simulink model "kondisi_genset_isolasi"  (R2024b)
settings: Solver=VariableStepAuto  StartTime=0.0  StopTime=10.0  RelTol=1e-3
undefined symbols (not defined in the file): D1, Delta
libraries: spsThreePhaseBreakerLib x36, spsThreePhaseParallelRLCLoadLib x35, spsThreePhaseTransformerTwoWindingsLib x18, spsThreePhasePISectionLineLib x14, spsExcitationSystemLib x13, spsSynchronousMachinepuStandardLib x13, spsGroundLib x4, spsThreePhaseParallelRLCBranchLib x4, spsThreePhaseVIMeasurementLib x4, spspowerguiLib x1
settings Model: Creator=irfan  LastModifiedBy=irfan

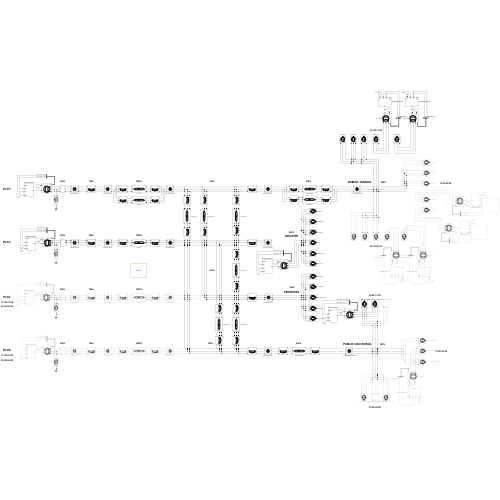
[thumbnail: Simulink's stored preview of the top-level diagram]
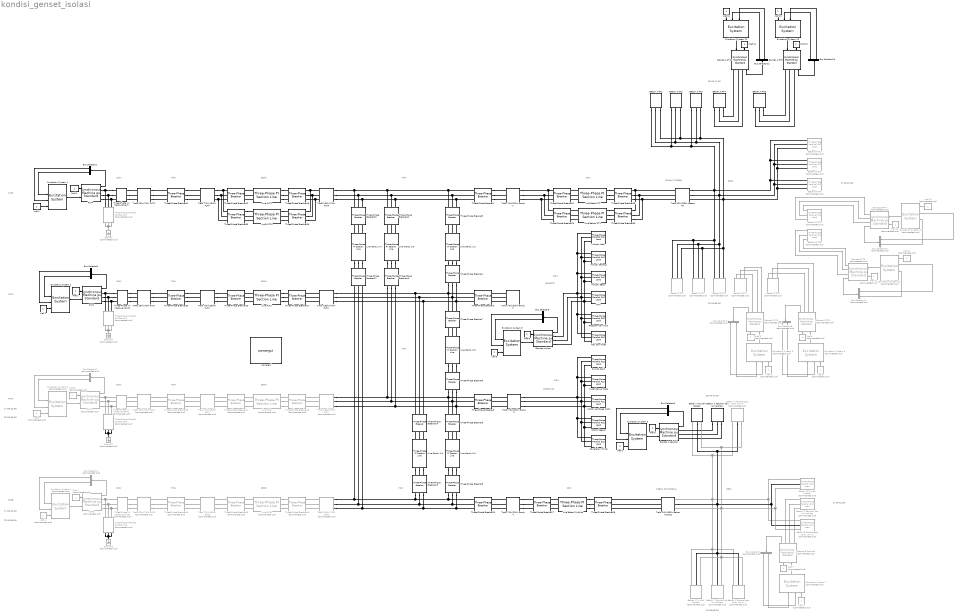
== system kondisi_genset_isolasi ==
  note: 05.00-17.00
  note: PLTP
  note: PLTU
  note: PLTA
  note: PLTB
  note: RUMAH TANGGA
  note: INDUSTRI
  note: PRIORITAS
  note: PUBLIK DAN SOSIAL
  note: 17.00-22.00
  note: 22.00-05.00
  note: 05.00-17.00
  note: 17.00-22.00
  note: 22.00-05.00
  note: 70kV
  note: 150kV
  note: 20kV
  note: 380V
  note: 380V
  note: 17.00-22.00
  note: 17.00-22.00
  note: 20kV
  note: 20kV
  note: 150kV
  note: 150kV
  note: 150kV
  note: 20kV
  note: 70kV
  note: 70kV
  note: 70kV
  note: 70kV
  note: 70kV
  note: 70kV
  note: 20kV
  note: 20kV
  note: 20kV
  note: 20kV
  note: 22.00-05.00
  note: 22.00-05.00
  Beban A Penerangan Jalan Umum : spsThreePhaseParallelRLCLoadLib/Three-Phase Parallel RLC Load  Commented=on  LConnTagsString=A|B|C  Configuration=Y (grounded)  NominalVoltage=380  Vabc=[1e3 1e3 1e3]  Vabcp=[1e3 1e3 1e3]  NominalFrequency=50  UnbalancedPower=off  ActivePower=0e6  InductivePower=0e6  CapacitivePower=0  Pabc=[10e3 9e3 11e3]  QLabc=[100 90 110]  QCabc=[100 90 110]  Pabcp=[10e3 9e3 11e3]  QLabcp=[100 90 110]  QCabcp=[100 90 110]  Measurements=Branch currents  LoadType=constant Z
  Beban A RT1 : spsThreePhaseParallelRLCLoadLib/Three-Phase Parallel RLC Load  LConnTagsString=A|B|C  Configuration=Y (grounded)  NominalVoltage=380  Vabc=[1e3 1e3 1e3]  Vabcp=[1e3 1e3 1e3]  NominalFrequency=50  UnbalancedPower=off  ActivePower=5.1e6  InductivePower=1.68e6  CapacitivePower=0  Pabc=[10e3 9e3 11e3]  QLabc=[100 90 110]  QCabc=[100 90 110]  Pabcp=[10e3 9e3 11e3]  QLabcp=[100 90 110]  QCabcp=[100 90 110]  Measurements=Branch currents  LoadType=constant Z
  Beban A RT2 : spsThreePhaseParallelRLCLoadLib/Three-Phase Parallel RLC Load  LConnTagsString=A|B|C  Configuration=Y (grounded)  NominalVoltage=380  Vabc=[1e3 1e3 1e3]  Vabcp=[1e3 1e3 1e3]  NominalFrequency=50  UnbalancedPower=off  ActivePower=8.06e6  InductivePower=2.65e6  CapacitivePower=0  Pabc=[10e3 9e3 11e3]  QLabc=[100 90 110]  QCabc=[100 90 110]  Pabcp=[10e3 9e3 11e3]  QLabcp=[100 90 110]  QCabcp=[100 90 110]  Measurements=Branch currents  LoadType=constant Z
  Beban A RT3 : spsThreePhaseParallelRLCLoadLib/Three-Phase Parallel RLC Load  LConnTagsString=A|B|C  Configuration=Y (grounded)  NominalVoltage=380  Vabc=[1e3 1e3 1e3]  Vabcp=[1e3 1e3 1e3]  NominalFrequency=50  UnbalancedPower=off  ActivePower=3e6  InductivePower=0.99e6  CapacitivePower=0  Pabc=[10e3 9e3 11e3]  QLabc=[100 90 110]  QCabc=[100 90 110]  Pabcp=[10e3 9e3 11e3]  QLabcp=[100 90 110]  QCabcp=[100 90 110]  Measurements=Branch currents  LoadType=constant Z
  Beban A RT4 : spsThreePhaseParallelRLCLoadLib/Three-Phase Parallel RLC Load  LConnTagsString=A|B|C  Configuration=Y (grounded)  NominalVoltage=380  Vabc=[1e3 1e3 1e3]  Vabcp=[1e3 1e3 1e3]  NominalFrequency=50  UnbalancedPower=off  ActivePower=1.5e6  InductivePower=0.49e6  CapacitivePower=0  Pabc=[10e3 9e3 11e3]  QLabc=[100 90 110]  QCabc=[100 90 110]  Pabcp=[10e3 9e3 11e3]  QLabcp=[100 90 110]  QCabcp=[100 90 110]  Measurements=Branch currents  LoadType=constant Z
  Beban A RT5 : spsThreePhaseParallelRLCLoadLib/Three-Phase Parallel RLC Load  LConnTagsString=A|B|C  Configuration=Y (grounded)  NominalVoltage=380  Vabc=[1e3 1e3 1e3]  Vabcp=[1e3 1e3 1e3]  NominalFrequency=50  UnbalancedPower=off  ActivePower=1.5e6  InductivePower=0.49e6  CapacitivePower=0  Pabc=[10e3 9e3 11e3]  QLabc=[100 90 110]  QCabc=[100 90 110]  Pabcp=[10e3 9e3 11e3]  QLabcp=[100 90 110]  QCabcp=[100 90 110]  Measurements=Branch currents  LoadType=constant Z
  Beban A Rumah Ibadah : spsThreePhaseParallelRLCLoadLib/Three-Phase Parallel RLC Load  LConnTagsString=A|B|C  Configuration=Y (grounded)  NominalVoltage=380  Vabc=[1e3 1e3 1e3]  Vabcp=[1e3 1e3 1e3]  NominalFrequency=50  UnbalancedPower=off  ActivePower=1.122e6  InductivePower=0.6954e6  CapacitivePower=0  Pabc=[10e3 9e3 11e3]  QLabc=[100 90 110]  QCabc=[100 90 110]  Pabcp=[10e3 9e3 11e3]  QLabcp=[100 90 110]  QCabcp=[100 90 110]  Measurements=Branch currents  LoadType=constant Z
  Beban A Sekolah dan Universitas : spsThreePhaseParallelRLCLoadLib/Three-Phase Parallel RLC Load  LConnTagsString=A|B|C  Configuration=Y (grounded)  NominalVoltage=380  Vabc=[1e3 1e3 1e3]  Vabcp=[1e3 1e3 1e3]  NominalFrequency=50  UnbalancedPower=off  ActivePower=0.85e6  InductivePower=0.5268e6  CapacitivePower=0  Pabc=[10e3 9e3 11e3]  QLabc=[100 90 110]  QCabc=[100 90 110]  Pabcp=[10e3 9e3 11e3]  QLabcp=[100 90 110]  QCabcp=[100 90 110]  Measurements=Branch currents  LoadType=constant Z
  Beban B Penerangan Jalan Umum : spsThreePhaseParallelRLCLoadLib/Three-Phase Parallel RLC Load  Commented=on  LConnTagsString=A|B|C  Configuration=Y (grounded)  NominalVoltage=380  Vabc=[1e3 1e3 1e3]  Vabcp=[1e3 1e3 1e3]  NominalFrequency=50  UnbalancedPower=off  ActivePower=1.7e6  InductivePower=1.0536e6  CapacitivePower=0  Pabc=[10e3 9e3 11e3]  QLabc=[100 90 110]  QCabc=[100 90 110]  Pabcp=[10e3 9e3 11e3]  QLabcp=[100 90 110]  QCabcp=[100 90 110]  Measurements=Branch currents  LoadType=constant Z
  Beban B RT1 : spsThreePhaseParallelRLCLoadLib/Three-Phase Parallel RLC Load  Commented=on  LConnTagsString=A|B|C  Configuration=Y (grounded)  NominalVoltage=380  Vabc=[1e3 1e3 1e3]  Vabcp=[1e3 1e3 1e3]  NominalFrequency=50  UnbalancedPower=off  ActivePower=21.93e6  InductivePower=7.21e6  CapacitivePower=0  Pabc=[10e3 9e3 11e3]  QLabc=[100 90 110]  QCabc=[100 90 110]  Pabcp=[10e3 9e3 11e3]  QLabcp=[100 90 110]  QCabcp=[100 90 110]  Measurements=Branch currents  LoadType=constant Z
  Beban B RT2 : spsThreePhaseParallelRLCLoadLib/Three-Phase Parallel RLC Load  Commented=on  LConnTagsString=A|B|C  Configuration=Y (grounded)  NominalVoltage=380  Vabc=[1e3 1e3 1e3]  Vabcp=[1e3 1e3 1e3]  NominalFrequency=50  UnbalancedPower=off  ActivePower=17.58e6  InductivePower=5.78e6  CapacitivePower=0  Pabc=[10e3 9e3 11e3]  QLabc=[100 90 110]  QCabc=[100 90 110]  Pabcp=[10e3 9e3 11e3]  QLabcp=[100 90 110]  QCabcp=[100 90 110]  Measurements=Branch currents  LoadType=constant Z
  Beban B RT3 : spsThreePhaseParallelRLCLoadLib/Three-Phase Parallel RLC Load  Commented=on  LConnTagsString=A|B|C  Configuration=Y (grounded)  NominalVoltage=380  Vabc=[1e3 1e3 1e3]  Vabcp=[1e3 1e3 1e3]  NominalFrequency=50  UnbalancedPower=off  ActivePower=6.53e6  InductivePower=2.14e6  CapacitivePower=0  Pabc=[10e3 9e3 11e3]  QLabc=[100 90 110]  QCabc=[100 90 110]  Pabcp=[10e3 9e3 11e3]  QLabcp=[100 90 110]  QCabcp=[100 90 110]  Measurements=Branch currents  LoadType=constant Z
  Beban B RT4 : spsThreePhaseParallelRLCLoadLib/Three-Phase Parallel RLC Load  Commented=on  LConnTagsString=A|B|C  Configuration=Y (grounded)  NominalVoltage=380  Vabc=[1e3 1e3 1e3]  Vabcp=[1e3 1e3 1e3]  NominalFrequency=50  UnbalancedPower=off  ActivePower=3.26e6  InductivePower=1.07e6  CapacitivePower=0  Pabc=[10e3 9e3 11e3]  QLabc=[100 90 110]  QCabc=[100 90 110]  Pabcp=[10e3 9e3 11e3]  QLabcp=[100 90 110]  QCabcp=[100 90 110]  Measurements=Branch currents  LoadType=constant Z
  Beban B RT5 : spsThreePhaseParallelRLCLoadLib/Three-Phase Parallel RLC Load  Commented=on  LConnTagsString=A|B|C  Configuration=Y (grounded)  NominalVoltage=380  Vabc=[1e3 1e3 1e3]  Vabcp=[1e3 1e3 1e3]  NominalFrequency=50  UnbalancedPower=off  ActivePower=2.91e6  InductivePower=0.96e6  CapacitivePower=0  Pabc=[10e3 9e3 11e3]  QLabc=[100 90 110]  QCabc=[100 90 110]  Pabcp=[10e3 9e3 11e3]  QLabcp=[100 90 110]  QCabcp=[100 90 110]  Measurements=Branch currents  LoadType=constant Z
  Beban B Rumah Ibadah : spsThreePhaseParallelRLCLoadLib/Three-Phase Parallel RLC Load  Commented=on  LConnTagsString=A|B|C  Configuration=Y (grounded)  NominalVoltage=380  Vabc=[1e3 1e3 1e3]  Vabcp=[1e3 1e3 1e3]  NominalFrequency=50  UnbalancedPower=off  ActivePower=1.122e6  InductivePower=0.6954e6  CapacitivePower=0  Pabc=[10e3 9e3 11e3]  QLabc=[100 90 110]  QCabc=[100 90 110]  Pabcp=[10e3 9e3 11e3]  QLabcp=[100 90 110]  QCabcp=[100 90 110]  Measurements=Branch currents  LoadType=constant Z
  Beban B Sekolah dan Universitas : spsThreePhaseParallelRLCLoadLib/Three-Phase Parallel RLC Load  Commented=on  LConnTagsString=A|B|C  Configuration=Y (grounded)  NominalVoltage=380  Vabc=[1e3 1e3 1e3]  Vabcp=[1e3 1e3 1e3]  NominalFrequency=50  UnbalancedPower=off  ActivePower=0.85e6  InductivePower=0.5268e6  CapacitivePower=0  Pabc=[10e3 9e3 11e3]  QLabc=[100 90 110]  QCabc=[100 90 110]  Pabcp=[10e3 9e3 11e3]  QLabcp=[100 90 110]  QCabcp=[100 90 110]  Measurements=Branch currents  LoadType=constant Z
  Beban C Penerangan Jalan Umum : spsThreePhaseParallelRLCLoadLib/Three-Phase Parallel RLC Load  Commented=on  LConnTagsString=A|B|C  Configuration=Y (grounded)  NominalVoltage=380  Vabc=[1e3 1e3 1e3]  Vabcp=[1e3 1e3 1e3]  NominalFrequency=50  UnbalancedPower=off  ActivePower=1.7e6  InductivePower=1.0536e6  CapacitivePower=0  Pabc=[10e3 9e3 11e3]  QLabc=[100 90 110]  QCabc=[100 90 110]  Pabcp=[10e3 9e3 11e3]  QLabcp=[100 90 110]  QCabcp=[100 90 110]  Measurements=Branch currents  LoadType=constant Z
  Beban C RT1 : spsThreePhaseParallelRLCLoadLib/Three-Phase Parallel RLC Load  Commented=on  LConnTagsString=A|B|C  Configuration=Y (grounded)  NominalVoltage=380  Vabc=[1e3 1e3 1e3]  Vabcp=[1e3 1e3 1e3]  NominalFrequency=50  UnbalancedPower=off  ActivePower=15.81e6  InductivePower=5.2e6  CapacitivePower=0  Pabc=[10e3 9e3 11e3]  QLabc=[100 90 110]  QCabc=[100 90 110]  Pabcp=[10e3 9e3 11e3]  QLabcp=[100 90 110]  QCabcp=[100 90 110]  Measurements=Branch currents  LoadType=constant Z
  Beban C RT2 : spsThreePhaseParallelRLCLoadLib/Three-Phase Parallel RLC Load  Commented=on  LConnTagsString=A|B|C  Configuration=Y (grounded)  NominalVoltage=380  Vabc=[1e3 1e3 1e3]  Vabcp=[1e3 1e3 1e3]  NominalFrequency=50  UnbalancedPower=off  ActivePower=13.71e6  InductivePower=4.51e6  CapacitivePower=0  Pabc=[10e3 9e3 11e3]  QLabc=[100 90 110]  QCabc=[100 90 110]  Pabcp=[10e3 9e3 11e3]  QLabcp=[100 90 110]  QCabcp=[100 90 110]  Measurements=Branch currents  LoadType=constant Z
  Beban C RT3 : spsThreePhaseParallelRLCLoadLib/Three-Phase Parallel RLC Load  Commented=on  LConnTagsString=A|B|C  Configuration=Y (grounded)  NominalVoltage=380  Vabc=[1e3 1e3 1e3]  Vabcp=[1e3 1e3 1e3]  NominalFrequency=50  UnbalancedPower=off  ActivePower=5.25e6  InductivePower=1.73e6  CapacitivePower=0  Pabc=[10e3 9e3 11e3]  QLabc=[100 90 110]  QCabc=[100 90 110]  Pabcp=[10e3 9e3 11e3]  QLabcp=[100 90 110]  QCabcp=[100 90 110]  Measurements=Branch currents  LoadType=constant Z
  Beban C RT4 : spsThreePhaseParallelRLCLoadLib/Three-Phase Parallel RLC Load  Commented=on  LConnTagsString=A|B|C  Configuration=Y (grounded)  NominalVoltage=380  Vabc=[1e3 1e3 1e3]  Vabcp=[1e3 1e3 1e3]  NominalFrequency=50  UnbalancedPower=off  ActivePower=2.86e6  InductivePower=0.94e6  CapacitivePower=0  Pabc=[10e3 9e3 11e3]  QLabc=[100 90 110]  QCabc=[100 90 110]  Pabcp=[10e3 9e3 11e3]  QLabcp=[100 90 110]  QCabcp=[100 90 110]  Measurements=Branch currents  LoadType=constant Z
  Beban C RT5 : spsThreePhaseParallelRLCLoadLib/Three-Phase Parallel RLC Load  Commented=on  LConnTagsString=A|B|C  Configuration=Y (grounded)  NominalVoltage=380  Vabc=[1e3 1e3 1e3]  Vabcp=[1e3 1e3 1e3]  NominalFrequency=50  UnbalancedPower=off  ActivePower=3.17e6  InductivePower=1.04e6  CapacitivePower=0  Pabc=[10e3 9e3 11e3]  QLabc=[100 90 110]  QCabc=[100 90 110]  Pabcp=[10e3 9e3 11e3]  QLabcp=[100 90 110]  QCabcp=[100 90 110]  Measurements=Branch currents  LoadType=constant Z
  Beban C Rumah Ibadah : spsThreePhaseParallelRLCLoadLib/Three-Phase Parallel RLC Load  Commented=on  LConnTagsString=A|B|C  Configuration=Y (grounded)  NominalVoltage=380  Vabc=[1e3 1e3 1e3]  Vabcp=[1e3 1e3 1e3]  NominalFrequency=50  UnbalancedPower=off  ActivePower=1.122e6  InductivePower=0.6954e6  CapacitivePower=0  Pabc=[10e3 9e3 11e3]  QLabc=[100 90 110]  QCabc=[100 90 110]  Pabcp=[10e3 9e3 11e3]  QLabcp=[100 90 110]  QCabcp=[100 90 110]  Measurements=Branch currents  LoadType=constant Z
  Beban C Sekolah dan Universitas : spsThreePhaseParallelRLCLoadLib/Three-Phase Parallel RLC Load  Commented=on  LConnTagsString=A|B|C  Configuration=Y (grounded)  NominalVoltage=380  Vabc=[1e3 1e3 1e3]  Vabcp=[1e3 1e3 1e3]  NominalFrequency=50  UnbalancedPower=off  ActivePower=0e6  InductivePower=0e6  CapacitivePower=0  Pabc=[10e3 9e3 11e3]  QLabc=[100 90 110]  QCabc=[100 90 110]  Pabcp=[10e3 9e3 11e3]  QLabcp=[100 90 110]  QCabcp=[100 90 110]  Measurements=Branch currents  LoadType=constant Z
  Bus Selector{1,3,5..6,12..13} (6 alike) : BusSelector  OutputSignals="dq0 components.Stator voltage  vd (pu),dq0 components.Stator voltage  vq (pu)"
  Bus Selector{2,4,7..11} (7 alike) : BusSelector  Commented=on  OutputSignals="dq0 components.Stator voltage  vd (pu),dq0 components.Stator voltage  vq (pu)"
  Excitation System 1 : spsExcitationSystemLib/Excitation System  tr=20e-3  reg=[ 300, 0.001 ]  exc=[ 1, 0 ]  tgr=[ 0, 0 ]  damp=[ 0.001, 0.1 ]  sat=[ 0, 0 ]  lim=[ -11.5, 11.5, 0 ]  v0=[1 2.6645]
      settings: LibrarySourceBlock=sps_lib/Electrical Machines/Synchronous Machine Control/Excitation System
  Excitation System {4,7..11} (6 alike) : spsExcitationSystemLib/Excitation System  Commented=on  tr=20e-3  reg=[ 300, 0.001 ]  exc=[ 1, 0 ]  tgr=[ 0, 0 ]  damp=[ 0.001, 0.1 ]  sat=[ 0, 0 ]  lim=[ -11.5, 11.5, 0 ]  v0=[0.99992 10.989]
      settings: LibrarySourceBlock=sps_lib/Electrical Machines/Synchronous Machine Control/Excitation System
  Excitation System {2,5..6,12..13} (5 alike) : spsExcitationSystemLib/Excitation System  tr=20e-3  reg=[ 300, 0.001 ]  exc=[ 1, 0 ]  tgr=[ 0, 0 ]  damp=[ 0.001, 0.1 ]  sat=[ 0, 0 ]  lim=[ -11.5, 11.5, 0 ]  v0=[0.99992 10.989]
      settings: LibrarySourceBlock=sps_lib/Electrical Machines/Synchronous Machine Control/Excitation System
  Excitation System 3 : spsExcitationSystemLib/Excitation System  Commented=on  tr=20e-3  reg=[ 300, 0.001 ]  exc=[ 1, 0 ]  tgr=[ 0, 0 ]  damp=[ 0.001, 0.1 ]  sat=[ 0, 0 ]  lim=[ -11.5, 11.5, 0 ]  v0=[1 2.6645]
      settings: LibrarySourceBlock=sps_lib/Electrical Machines/Synchronous Machine Control/Excitation System
  Genset A RT4 : spsSynchronousMachinepuStandardLib/Synchronous Machine pu Standard  PresetModel=No  MechanicalLoad=Mechanical power Pm  ShowDetailedParameters=on  RotorType=Salient-pole  Units=per unit standard parameters  MeasurementBus=off  NominalParameters=[1.5789e6 380 50]  Reactances1=[ 1.81, 0.3, 0.23, 1.76, 0.65, 0.25, 0.15 ]  Reactances2=[2.24 0.17 0.12 1.02 0.13 0.1]  dAxisTimeConstants=Short-circuit  qAxisTimeConstants=Short-circuit  TimeConstants1="[ 4.4849  0.0681  0.1  ]"  TimeConstants2=[ 8.0, 0.03, 1.0, 0.07 ]  TimeConstants3="[  4.49  0.0681  0.0513  ]"  TimeConstants4=[ 8.0, 0.03, 0.3371, 0.0295 ]  TimeConstants5=[ 1.01, 0.053, 0.1 ]  TimeConstants6=[ 1.3201, 0.023, 1.0, 0.07 ]  TimeConstants7=[0.012 0.003 0.003]  TimeConstants8=[ 1.3201, 0.0231, 0.3371, 0.0295 ]  StatorResistance=0.037875  Mechanical=[0.1028 0.02056 2]  PolePairs=20  InitialConditions="[ 0  0  0  0  0  0  0  0  1 ]"  SetSaturation=on  Saturation=[0.6404,0.7127,0.8441,0.9214,0.9956,1.082,1.19,1.316,1.457;0.7,0.7698,0.8872,0.9466,0.9969,1.046,1.1,1.151,1.201]  LoadFlowParameters=[1,0,0,0,0]  TsPowergui=0  TsBlock=-1  IterativeModel=Trapezoidal non iterative  IterativeDiscreteModel=Trapezoidal non iterative  BusType=swing  Pref=1.5e6  Qref=0.49e6  Qmin=-inf  Qmax=inf  PLF=0  QLF=0
  Genset A RT5 : spsSynchronousMachinepuStandardLib/Synchronous Machine pu Standard  PresetModel=No  MechanicalLoad=Mechanical power Pm  ShowDetailedParameters=on  RotorType=Salient-pole  Units=per unit standard parameters  MeasurementBus=off  NominalParameters=[1.5789e6 380 50]  Reactances1=[ 1.81, 0.3, 0.23, 1.76, 0.65, 0.25, 0.15 ]  Reactances2=[2.24 0.17 0.12 1.02 0.13 0.1]  dAxisTimeConstants=Short-circuit  qAxisTimeConstants=Short-circuit  TimeConstants1="[ 4.4849  0.0681  0.1  ]"  TimeConstants2=[ 8.0, 0.03, 1.0, 0.07 ]  TimeConstants3="[  4.49  0.0681  0.0513  ]"  TimeConstants4=[ 8.0, 0.03, 0.3371, 0.0295 ]  TimeConstants5=[ 1.01, 0.053, 0.1 ]  TimeConstants6=[ 1.3201, 0.023, 1.0, 0.07 ]  TimeConstants7=[0.012 0.003 0.003]  TimeConstants8=[ 1.3201, 0.0231, 0.3371, 0.0295 ]  StatorResistance=0.037875  Mechanical=[0.1028 0.02056 2]  PolePairs=20  InitialConditions="[ 0  0  0  0  0  0  0  0  1 ]"  SetSaturation=on  Saturation=[0.6404,0.7127,0.8441,0.9214,0.9956,1.082,1.19,1.316,1.457;0.7,0.7698,0.8872,0.9466,0.9969,1.046,1.1,1.151,1.201]  LoadFlowParameters=[1,0,0,0,0]  TsPowergui=0  TsBlock=-1  IterativeModel=Trapezoidal non iterative  IterativeDiscreteModel=Trapezoidal non iterative  BusType=swing  Pref=1.5e6  Qref=0.49e6  Qmin=-inf  Qmax=inf  PLF=0  QLF=0
  Genset A Sekolah : spsSynchronousMachinepuStandardLib/Synchronous Machine pu Standard  PresetModel=No  MechanicalLoad=Mechanical power Pm  ShowDetailedParameters=on  RotorType=Salient-pole  Units=per unit standard parameters  MeasurementBus=off  NominalParameters=[1.0000e6 380 50]  Reactances1=[ 1.81, 0.3, 0.23, 1.76, 0.65, 0.25, 0.15 ]  Reactances2=[2.24 0.17 0.12 1.02 0.13 0.1]  dAxisTimeConstants=Short-circuit  qAxisTimeConstants=Short-circuit  TimeConstants1="[ 4.4849  0.0681  0.1  ]"  TimeConstants2=[ 8.0, 0.03, 1.0, 0.07 ]  TimeConstants3="[  4.49  0.0681  0.0513  ]"  TimeConstants4=[ 8.0, 0.03, 0.3371, 0.0295 ]  TimeConstants5=[ 1.01, 0.053, 0.1 ]  TimeConstants6=[ 1.3201, 0.023, 1.0, 0.07 ]  TimeConstants7=[0.012 0.003 0.003]  TimeConstants8=[ 1.3201, 0.0231, 0.3371, 0.0295 ]  StatorResistance=0.037875  Mechanical=[0.1028 0.02056 2]  PolePairs=20  InitialConditions="[ 0  0  0  0  0  0  0  0  1 ]"  SetSaturation=on  Saturation=[0.6404,0.7127,0.8441,0.9214,0.9956,1.082,1.19,1.316,1.457;0.7,0.7698,0.8872,0.9466,0.9969,1.046,1.1,1.151,1.201]  LoadFlowParameters=[1,0,0,0,0]  TsPowergui=0  TsBlock=-1  IterativeModel=Trapezoidal non iterative  IterativeDiscreteModel=Trapezoidal non iterative  BusType=swing  Pref=0.85e6  Qref=0.5268e6  Qmin=-inf  Qmax=inf  PLF=0  QLF=0
  Genset B RT4 : spsSynchronousMachinepuStandardLib/Synchronous Machine pu Standard  Commented=on  PresetModel=No  MechanicalLoad=Mechanical power Pm  ShowDetailedParameters=on  RotorType=Salient-pole  Units=per unit standard parameters  MeasurementBus=off  NominalParameters=[3.4342e6 380 50]  Reactances1=[ 1.81, 0.3, 0.23, 1.76, 0.65, 0.25, 0.15 ]  Reactances2=[2.24 0.17 0.12 1.02 0.13 0.1]  dAxisTimeConstants=Short-circuit  qAxisTimeConstants=Short-circuit  TimeConstants1="[ 4.4849  0.0681  0.1  ]"  TimeConstants2=[ 8.0, 0.03, 1.0, 0.07 ]  TimeConstants3="[  4.49  0.0681  0.0513  ]"  TimeConstants4=[ 8.0, 0.03, 0.3371, 0.0295 ]  TimeConstants5=[ 1.01, 0.053, 0.1 ]  TimeConstants6=[ 1.3201, 0.023, 1.0, 0.07 ]  TimeConstants7=[0.012 0.003 0.003]  TimeConstants8=[ 1.3201, 0.0231, 0.3371, 0.0295 ]  StatorResistance=0.037875  Mechanical=[0.1028 0.02056 2]  PolePairs=20  InitialConditions="[ 0  0  0  0  0  0  0  0  1 ]"  SetSaturation=on  Saturation=[0.6404,0.7127,0.8441,0.9214,0.9956,1.082,1.19,1.316,1.457;0.7,0.7698,0.8872,0.9466,0.9969,1.046,1.1,1.151,1.201]  LoadFlowParameters=[1,0,0,0,0]  TsPowergui=0  TsBlock=-1  IterativeModel=Trapezoidal non iterative  IterativeDiscreteModel=Trapezoidal non iterative  BusType=swing  Pref=3.26e6  Qref=1.07e6  Qmin=-inf  Qmax=inf  PLF=0  QLF=0
  Genset B RT5 : spsSynchronousMachinepuStandardLib/Synchronous Machine pu Standard  Commented=on  PresetModel=No  MechanicalLoad=Mechanical power Pm  ShowDetailedParameters=on  RotorType=Salient-pole  Units=per unit standard parameters  MeasurementBus=off  NominalParameters=[3.0632e6 380 50]  Reactances1=[ 1.81, 0.3, 0.23, 1.76, 0.65, 0.25, 0.15 ]  Reactances2=[2.24 0.17 0.12 1.02 0.13 0.1]  dAxisTimeConstants=Short-circuit  qAxisTimeConstants=Short-circuit  TimeConstants1="[ 4.4849  0.0681  0.1  ]"  TimeConstants2=[ 8.0, 0.03, 1.0, 0.07 ]  TimeConstants3="[  4.49  0.0681  0.0513  ]"  TimeConstants4=[ 8.0, 0.03, 0.3371, 0.0295 ]  TimeConstants5=[ 1.01, 0.053, 0.1 ]  TimeConstants6=[ 1.3201, 0.023, 1.0, 0.07 ]  TimeConstants7=[0.012 0.003 0.003]  TimeConstants8=[ 1.3201, 0.0231, 0.3371, 0.0295 ]  StatorResistance=0.037875  Mechanical=[0.1028 0.02056 2]  PolePairs=20  InitialConditions="[ 0  0  0  0  0  0  0  0  1 ]"  SetSaturation=on  Saturation=[0.6404,0.7127,0.8441,0.9214,0.9956,1.082,1.19,1.316,1.457;0.7,0.7698,0.8872,0.9466,0.9969,1.046,1.1,1.151,1.201]  LoadFlowParameters=[1,0,0,0,0]  TsPowergui=0  TsBlock=-1  IterativeModel=Trapezoidal non iterative  IterativeDiscreteModel=Trapezoidal non iterative  BusType=swing  Pref=2.91e6  Qref=0.96e6  Qmin=-inf  Qmax=inf  PLF=0  QLF=0
  Genset B Sekolah : spsSynchronousMachinepuStandardLib/Synchronous Machine pu Standard  Commented=on  PresetModel=No  MechanicalLoad=Mechanical power Pm  ShowDetailedParameters=on  RotorType=Salient-pole  Units=per unit standard parameters  MeasurementBus=off  NominalParameters=[1e6 380 50]  Reactances1=[ 1.81, 0.3, 0.23, 1.76, 0.65, 0.25, 0.15 ]  Reactances2=[2.24 0.17 0.12 1.02 0.13 0.1]  dAxisTimeConstants=Short-circuit  qAxisTimeConstants=Short-circuit  TimeConstants1="[ 4.4849  0.0681  0.1  ]"  TimeConstants2=[ 8.0, 0.03, 1.0, 0.07 ]  TimeConstants3="[  4.49  0.0681  0.0513  ]"  TimeConstants4=[ 8.0, 0.03, 0.3371, 0.0295 ]  TimeConstants5=[ 1.01, 0.053, 0.1 ]  TimeConstants6=[ 1.3201, 0.023, 1.0, 0.07 ]  TimeConstants7=[0.012 0.003 0.003]  TimeConstants8=[ 1.3201, 0.0231, 0.3371, 0.0295 ]  StatorResistance=0.037875  Mechanical=[0.1028 0.02056 2]  PolePairs=20  InitialConditions="[ 0  0  0  0  0  0  0  0  1 ]"  SetSaturation=on  Saturation=[0.6404,0.7127,0.8441,0.9214,0.9956,1.082,1.19,1.316,1.457;0.7,0.7698,0.8872,0.9466,0.9969,1.046,1.1,1.151,1.201]  LoadFlowParameters=[1,0,0,0,0]  TsPowergui=0  TsBlock=-1  IterativeModel=Trapezoidal non iterative  IterativeDiscreteModel=Trapezoidal non iterative  BusType=swing  Pref=0.85e6  Qref=0.5268e6  Qmin=-inf  Qmax=inf  PLF=0  QLF=0
  Genset C RT4 : spsSynchronousMachinepuStandardLib/Synchronous Machine pu Standard  Commented=on  PresetModel=No  MechanicalLoad=Mechanical power Pm  ShowDetailedParameters=on  RotorType=Salient-pole  Units=per unit standard parameters  MeasurementBus=off  NominalParameters=[3.0132e6 380 50]  Reactances1=[ 1.81, 0.3, 0.23, 1.76, 0.65, 0.25, 0.15 ]  Reactances2=[2.24 0.17 0.12 1.02 0.13 0.1]  dAxisTimeConstants=Short-circuit  qAxisTimeConstants=Short-circuit  TimeConstants1="[ 4.4849  0.0681  0.1  ]"  TimeConstants2=[ 8.0, 0.03, 1.0, 0.07 ]  TimeConstants3="[  4.49  0.0681  0.0513  ]"  TimeConstants4=[ 8.0, 0.03, 0.3371, 0.0295 ]  TimeConstants5=[ 1.01, 0.053, 0.1 ]  TimeConstants6=[ 1.3201, 0.023, 1.0, 0.07 ]  TimeConstants7=[0.012 0.003 0.003]  TimeConstants8=[ 1.3201, 0.0231, 0.3371, 0.0295 ]  StatorResistance=0.037875  Mechanical=[0.1028 0.02056 2]  PolePairs=20  InitialConditions="[ 0  0  0  0  0  0  0  0  1 ]"  SetSaturation=on  Saturation=[0.6404,0.7127,0.8441,0.9214,0.9956,1.082,1.19,1.316,1.457;0.7,0.7698,0.8872,0.9466,0.9969,1.046,1.1,1.151,1.201]  LoadFlowParameters=[1,0,0,0,0]  TsPowergui=0  TsBlock=-1  IterativeModel=Trapezoidal non iterative  IterativeDiscreteModel=Trapezoidal non iterative  BusType=swing  Pref=2.86e6  Qref=0.94e6  Qmin=-inf  Qmax=inf  PLF=0  QLF=0
  Genset C RT5 : spsSynchronousMachinepuStandardLib/Synchronous Machine pu Standard  Commented=on  PresetModel=No  MechanicalLoad=Mechanical power Pm  ShowDetailedParameters=on  RotorType=Salient-pole  Units=per unit standard parameters  MeasurementBus=off  NominalParameters=[3.3316e6 380 50]  Reactances1=[ 1.81, 0.3, 0.23, 1.76, 0.65, 0.25, 0.15 ]  Reactances2=[2.24 0.17 0.12 1.02 0.13 0.1]  dAxisTimeConstants=Short-circuit  qAxisTimeConstants=Short-circuit  TimeConstants1="[ 4.4849  0.0681  0.1  ]"  TimeConstants2=[ 8.0, 0.03, 1.0, 0.07 ]  TimeConstants3="[  4.49  0.0681  0.0513  ]"  TimeConstants4=[ 8.0, 0.03, 0.3371, 0.0295 ]  TimeConstants5=[ 1.01, 0.053, 0.1 ]  TimeConstants6=[ 1.3201, 0.023, 1.0, 0.07 ]  TimeConstants7=[0.012 0.003 0.003]  TimeConstants8=[ 1.3201, 0.0231, 0.3371, 0.0295 ]  StatorResistance=0.037875  Mechanical=[0.1028 0.02056 2]  PolePairs=20  InitialConditions="[ 0  0  0  0  0  0  0  0  1 ]"  SetSaturation=on  Saturation=[0.6404,0.7127,0.8441,0.9214,0.9956,1.082,1.19,1.316,1.457;0.7,0.7698,0.8872,0.9466,0.9969,1.046,1.1,1.151,1.201]  LoadFlowParameters=[1,0,0,0,0]  TsPowergui=0  TsBlock=-1  IterativeModel=Trapezoidal non iterative  IterativeDiscreteModel=Trapezoidal non iterative  BusType=swing  Pref=3.17e6  Qref=1.04e6  Qmin=-inf  Qmax=inf  PLF=0  QLF=0
  Genset Industri : spsSynchronousMachinepuStandardLib/Synchronous Machine pu Standard  PresetModel=No  MechanicalLoad=Mechanical power Pm  ShowDetailedParameters=on  RotorType=Salient-pole  Units=per unit standard parameters  MeasurementBus=off  NominalParameters=[79.1000e6 20e3 50]  Reactances1=[ 1.81, 0.3, 0.23, 1.76, 0.65, 0.25, 0.15 ]  Reactances2=[2.24 0.17 0.12 1.02 0.13 0.1]  dAxisTimeConstants=Short-circuit  qAxisTimeConstants=Short-circuit  TimeConstants1="[ 4.4849  0.0681  0.1  ]"  TimeConstants2=[ 8.0, 0.03, 1.0, 0.07 ]  TimeConstants3="[  4.49  0.0681  0.0513  ]"  TimeConstants4=[ 8.0, 0.03, 0.3371, 0.0295 ]  TimeConstants5=[ 1.01, 0.053, 0.1 ]  TimeConstants6=[ 1.3201, 0.023, 1.0, 0.07 ]  TimeConstants7=[0.012 0.003 0.003]  TimeConstants8=[ 1.3201, 0.0231, 0.3371, 0.0295 ]  StatorResistance=0.037875  Mechanical=[0.1028 0.02056 2]  PolePairs=20  InitialConditions="[ 0  0  0  0  0  0  0  0  1 ]"  SetSaturation=on  Saturation=[0.6404,0.7127,0.8441,0.9214,0.9956,1.082,1.19,1.316,1.457;0.7,0.7698,0.8872,0.9466,0.9969,1.046,1.1,1.151,1.201]  LoadFlowParameters=[1,0,0,0,0]  TsPowergui=0  TsBlock=-1  IterativeModel=Trapezoidal non iterative  IterativeDiscreteModel=Trapezoidal non iterative  BusType=swing  Pref=71.248e6  Qref=34.0616e6  Qmin=-inf  Qmax=inf  PLF=0  QLF=0
  Ground{,1..3} (4 alike) : spsGroundLib/Ground  Commented=on  LConnTagsString=a
  Industri Besar : spsThreePhaseParallelRLCLoadLib/Three-Phase Parallel RLC Load  LConnTagsString=A|B|C  Configuration=Y (grounded)  NominalVoltage=20e3  Vabc=[1e3 1e3 1e3]  Vabcp=[1e3 1e3 1e3]  NominalFrequency=50  UnbalancedPower=off  ActivePower=9.5e6  InductivePower=3.1225e6  CapacitivePower=0  Pabc=[10e3 9e3 11e3]  QLabc=[100 90 110]  QCabc=[100 90 110]  Pabcp=[10e3 9e3 11e3]  QLabcp=[100 90 110]  QCabcp=[100 90 110]  Measurements=Branch currents  LoadType=constant Z
  Industri Kecil : spsThreePhaseParallelRLCLoadLib/Three-Phase Parallel RLC Load  LConnTagsString=A|B|C  Configuration=Y (grounded)  NominalVoltage=20e3  Vabc=[1e3 1e3 1e3]  Vabcp=[1e3 1e3 1e3]  NominalFrequency=50  UnbalancedPower=off  ActivePower=5.808e6  InductivePower=3.1348e6  CapacitivePower=0  Pabc=[10e3 9e3 11e3]  QLabc=[100 90 110]  QCabc=[100 90 110]  Pabcp=[10e3 9e3 11e3]  QLabcp=[100 90 110]  QCabcp=[100 90 110]  Measurements=Branch currents  LoadType=constant Z
  Industri Sedang : spsThreePhaseParallelRLCLoadLib/Three-Phase Parallel RLC Load  LConnTagsString=A|B|C  Configuration=Y (grounded)  NominalVoltage=20e3  Vabc=[1e3 1e3 1e3]  Vabcp=[1e3 1e3 1e3]  NominalFrequency=50  UnbalancedPower=off  ActivePower=45e6  InductivePower=21.7945e6  CapacitivePower=0  Pabc=[10e3 9e3 11e3]  QLabc=[100 90 110]  QCabc=[100 90 110]  Pabcp=[10e3 9e3 11e3]  QLabcp=[100 90 110]  QCabcp=[100 90 110]  Measurements=Branch currents  LoadType=constant Z
  Istana Negara : spsThreePhaseParallelRLCLoadLib/Three-Phase Parallel RLC Load  LConnTagsString=A|B|C  Configuration=Y (grounded)  NominalVoltage=20e3  Vabc=[1e3 1e3 1e3]  Vabcp=[1e3 1e3 1e3]  NominalFrequency=50  UnbalancedPower=off  ActivePower=0.9e6  InductivePower=0.4359e6  CapacitivePower=0  Pabc=[10e3 9e3 11e3]  QLabc=[100 90 110]  QCabc=[100 90 110]  Pabcp=[10e3 9e3 11e3]  QLabcp=[100 90 110]  QCabcp=[100 90 110]  Measurements=Branch currents  LoadType=constant Z
  Kantor Lembaga Data : spsThreePhaseParallelRLCLoadLib/Three-Phase Parallel RLC Load  LConnTagsString=A|B|C  Configuration=Y (grounded)  NominalVoltage=20e3  Vabc=[1e3 1e3 1e3]  Vabcp=[1e3 1e3 1e3]  NominalFrequency=50  UnbalancedPower=off  ActivePower=0.9e6  InductivePower=0.4359e6  CapacitivePower=0  Pabc=[10e3 9e3 11e3]  QLabc=[100 90 110]  QCabc=[100 90 110]  Pabcp=[10e3 9e3 11e3]  QLabcp=[100 90 110]  QCabcp=[100 90 110]  Measurements=Branch currents  LoadType=constant Z
  Line Beban PubSos : spsThreePhasePISectionLineLib/Three-Phase PI Section Line  LConnTagsString=a|b|c  RConnTagsString=A|B|C  Length=3  Frequency=50  Resistances=[ 0.2530 0.3864]  Inductances="[ 0.5530e-3  4.1264e-3]"  Capacitances=[0.2060e-6 7.751e-9]
  Line Beban RT : spsThreePhasePISectionLineLib/Three-Phase PI Section Line  LConnTagsString=a|b|c  RConnTagsString=A|B|C  Length=3  Frequency=50  Resistances=[ 0.2530 0.3864]  Inductances="[ 0.5530e-3  4.1264e-3]"  Capacitances=[0.2060e-6 7.751e-9]
  Line Beban RT1 : spsThreePhasePISectionLineLib/Three-Phase PI Section Line  LConnTagsString=a|b|c  RConnTagsString=A|B|C  Length=3  Frequency=50  Resistances=[ 0.2530 0.3864]  Inductances="[ 0.5530e-3  4.1264e-3]"  Capacitances=[0.2060e-6 7.751e-9]
  Line Gardu 1-2 : spsThreePhasePISectionLineLib/Three-Phase PI Section Line  LConnTagsString=a|b|c  RConnTagsString=A|B|C  Length=20  Frequency=50  Resistances=[ 0.0605 0.3864]  Inductances="[ 0.6210e-3  4.1264e-3]"  Capacitances=[12.74e-9 7.751e-9]
  Line Gardu 1-3 : spsThreePhasePISectionLineLib/Three-Phase PI Section Line  LConnTagsString=a|b|c  RConnTagsString=A|B|C  Length=5  Frequency=50  Resistances=[ 0.0605 0.3864]  Inductances="[ 0.6210e-3  4.1264e-3]"  Capacitances=[12.74e-9 7.751e-9]
  Line Gardu 1-4 : spsThreePhasePISectionLineLib/Three-Phase PI Section Line  LConnTagsString=a|b|c  RConnTagsString=A|B|C  Length=20  Frequency=50  Resistances=[ 0.0605 0.3864]  Inductances="[ 0.6210e-3  4.1264e-3]"  Capacitances=[12.74e-9 7.751e-9]
  Line Gardu 2-3 : spsThreePhasePISectionLineLib/Three-Phase PI Section Line  LConnTagsString=a|b|c  RConnTagsString=A|B|C  Length=5  Frequency=50  Resistances=[ 0.0605 0.3864]  Inductances="[ 0.6210e-3  4.1264e-3]"  Capacitances=[12.74e-9 7.751e-9]
  Line Gardu 2-4 : spsThreePhasePISectionLineLib/Three-Phase PI Section Line  LConnTagsString=a|b|c  RConnTagsString=A|B|C  Length=20  Frequency=50  Resistances=[ 0.0605 0.3864]  Inductances="[ 0.0012  0.0035]"  Capacitances=[12.74e-9 7.751e-9]
  Line Gardu 3-4 : spsThreePhasePISectionLineLib/Three-Phase PI Section Line  LConnTagsString=a|b|c  RConnTagsString=A|B|C  Length=5  Frequency=50  Resistances=[ 0.0605 0.3864]  Inductances="[ 0.6210e-3  4.1264e-3]"  Capacitances=[12.74e-9 7.751e-9]
  Line PLTA : spsThreePhasePISectionLineLib/Three-Phase PI Section Line  Commented=on  LConnTagsString=a|b|c  RConnTagsString=A|B|C  Length=50  Frequency=50  Resistances=[ 0.0605 0.3864]  Inductances="[ 0.6210e-3  4.1264e-3]"  Capacitances=[12.74e-9 7.751e-9]
  Line PLTB : spsThreePhasePISectionLineLib/Three-Phase PI Section Line  Commented=on  LConnTagsString=a|b|c  RConnTagsString=A|B|C  Length=20  Frequency=50  Resistances=[ 0.0605 0.3864]  Inductances="[ 0.6210e-3  4.1264e-3]"  Capacitances=[0.149e-6 5e-9]
  Line PLTP : spsThreePhasePISectionLineLib/Three-Phase PI Section Line  LConnTagsString=a|b|c  RConnTagsString=A|B|C  Length=100  Frequency=50  Resistances=[ 0.0605 0.3864]  Inductances="[ 0.6210e-3  4.1264e-3]"  Capacitances=[12.74e-9 7.751e-9]
  Line PLTP1 : spsThreePhasePISectionLineLib/Three-Phase PI Section Line  LConnTagsString=a|b|c  RConnTagsString=A|B|C  Length=100  Frequency=50  Resistances=[ 0.0605 0.3864]  Inductances="[ 0.6210e-3  4.1264e-3]"  Capacitances=[12.74e-9 7.751e-9]
  Line PLTU : spsThreePhasePISectionLineLib/Three-Phase PI Section Line  LConnTagsString=a|b|c  RConnTagsString=A|B|C  Length=100  Frequency=50  Resistances=[ 0.0605 0.3864]  Inductances="[ 0.6210e-3  4.1264e-3]"  Capacitances=[12.74e-9 7.751e-9]
  Mall dan Hotel : spsThreePhaseParallelRLCLoadLib/Three-Phase Parallel RLC Load  LConnTagsString=A|B|C  Configuration=Y (grounded)  NominalVoltage=20e3  Vabc=[1e3 1e3 1e3]  Vabcp=[1e3 1e3 1e3]  NominalFrequency=50  UnbalancedPower=off  ActivePower=0.84e6  InductivePower=0.5426e6  CapacitivePower=0  Pabc=[10e3 9e3 11e3]  QLabc=[100 90 110]  QCabc=[100 90 110]  Pabcp=[10e3 9e3 11e3]  QLabcp=[100 90 110]  QCabcp=[100 90 110]  Measurements=Branch currents  LoadType=constant Z
  PLTA : spsSynchronousMachinepuStandardLib/Synchronous Machine pu Standard  Commented=on  PresetModel=No  MechanicalLoad=Mechanical power Pm  ShowDetailedParameters=on  RotorType=Salient-pole  Units=per unit standard parameters  MeasurementBus=off  NominalParameters=[35.294e6 20e3 50]  Reactances1=[ 1.81, 0.3, 0.23, 1.76, 0.65, 0.25, 0.15 ]  Reactances2=[2.24 0.17 0.12 1.02 0.13 0.1]  dAxisTimeConstants=Short-circuit  qAxisTimeConstants=Short-circuit  TimeConstants1="[ 4.4849  0.0681  0.1  ]"  TimeConstants2=[ 8.0, 0.03, 1.0, 0.07 ]  TimeConstants3="[  4.49  0.0681  0.0513  ]"  TimeConstants4=[ 8.0, 0.03, 0.3371, 0.0295 ]  TimeConstants5=[ 1.01, 0.053, 0.1 ]  TimeConstants6=[ 1.3201, 0.023, 1.0, 0.07 ]  TimeConstants7=[0.012 0.003 0.003]  TimeConstants8=[ 1.3201, 0.0231, 0.3371, 0.0295 ]  StatorResistance=0.037875  Mechanical=[0.1028 0.02056 2]  PolePairs=20  InitialConditions=[0 -71.9687 0.82866 0.82866 0.82866 -48.3753 -168.375 71.6247 2.66449]  SetSaturation=on  Saturation=[0.6404,0.7127,0.8441,0.9214,0.9956,1.082,1.19,1.316,1.457;0.7,0.7698,0.8872,0.9466,0.9969,1.046,1.1,1.151,1.201]  LoadFlowParameters=[1,0,0,0,0]  TsPowergui=0  TsBlock=-1  IterativeModel=Trapezoidal non iterative  IterativeDiscreteModel=Trapezoidal non iterative  BusType=swing  Pref=30e6  Qref=0  Qmin=-Inf  Qmax=Inf  PLF=0  QLF=0
  PLTB : spsSynchronousMachinepuStandardLib/Synchronous Machine pu Standard  Commented=on  PresetModel=No  MechanicalLoad=Mechanical power Pm  ShowDetailedParameters=on  RotorType=Salient-pole  Units=per unit standard parameters  MeasurementBus=off  NominalParameters=[11.765e6 20e3 50]  Reactances1=[ 1.81, 0.3, 0.23, 1.76, 0.65, 0.25, 0.15 ]  Reactances2=[2.24 0.17 0.12 1.02 0.13 0.1]  dAxisTimeConstants=Short-circuit  qAxisTimeConstants=Short-circuit  TimeConstants1="[ 4.4849  0.0681  0.1  ]"  TimeConstants2=[ 8.0, 0.03, 1.0, 0.07 ]  TimeConstants3="[  4.49  0.0681  0.0513  ]"  TimeConstants4=[ 8.0, 0.03, 0.3371, 0.0295 ]  TimeConstants5=[ 1.01, 0.053, 0.1 ]  TimeConstants6=[ 1.3201, 0.023, 1.0, 0.07 ]  TimeConstants7=[0.012 0.003 0.003]  TimeConstants8=[ 1.3201, 0.0231, 0.3371, 0.0295 ]  StatorResistance=0.037875  Mechanical=[0.1028 0.02056 2]  PolePairs=20  InitialConditions="[ 0  0  0  0  0  0  0  0  1 ]"  SetSaturation=on  Saturation=[0.6404,0.7127,0.8441,0.9214,0.9956,1.082,1.19,1.316,1.457;0.7,0.7698,0.8872,0.9466,0.9969,1.046,1.1,1.151,1.201]  LoadFlowParameters=[1,0,0,0,0]  TsPowergui=0  TsBlock=-1  IterativeModel=Trapezoidal non iterative  IterativeDiscreteModel=Trapezoidal non iterative  BusType=PV  Pref=10e6  Qref=0  Qmin=-inf  Qmax=inf  PLF=0  QLF=0
  PLTP : spsSynchronousMachinepuStandardLib/Synchronous Machine pu Standard  PresetModel=No  MechanicalLoad=Mechanical power Pm  ShowDetailedParameters=on  RotorType=Salient-pole  Units=per unit standard parameters  MeasurementBus=off  NominalParameters=[94.12e6 20e3 50]  Reactances1=[ 1.81, 0.3, 0.23, 1.76, 0.65, 0.25, 0.15 ]  Reactances2=[2.24 0.17 0.12 1.02 0.13 0.1]  dAxisTimeConstants=Short-circuit  qAxisTimeConstants=Short-circuit  TimeConstants1="[ 4.4849  0.0681  0.1  ]"  TimeConstants2=[ 8.0, 0.03, 1.0, 0.07 ]  TimeConstants3="[  4.49  0.0681  0.0513  ]"  TimeConstants4=[ 8.0, 0.03, 0.3371, 0.0295 ]  TimeConstants5=[ 1.01, 0.053, 0.1 ]  TimeConstants6=[ 1.3201, 0.023, 1.0, 0.07 ]  TimeConstants7=[0.012 0.003 0.003]  TimeConstants8=[ 1.3201, 0.0231, 0.3371, 0.0295 ]  StatorResistance=0.037875  Mechanical=[0.1028 0.02056 2]  PolePairs=20  InitialConditions=[0 -71.9687 0.82866 0.82866 0.82866 -48.3753 -168.375 71.6247 2.66449]  SetSaturation=on  Saturation=[0.6404,0.7127,0.8441,0.9214,0.9956,1.082,1.19,1.316,1.457;0.7,0.7698,0.8872,0.9466,0.9969,1.046,1.1,1.151,1.201]  LoadFlowParameters=[1,0,0,0,0]  TsPowergui=0  TsBlock=-1  IterativeModel=Trapezoidal non iterative  IterativeDiscreteModel=Trapezoidal non iterative  BusType=swing  Pref=80e6  Qref=0  Qmin=-Inf  Qmax=Inf  PLF=0  QLF=0
  PLTU : spsSynchronousMachinepuStandardLib/Synchronous Machine pu Standard  PresetModel=No  MechanicalLoad=Mechanical power Pm  ShowDetailedParameters=on  RotorType=Salient-pole  Units=per unit standard parameters  MeasurementBus=off  NominalParameters=[117.65e6 20e3 50]  Reactances1=[ 1.81, 0.3, 0.23, 1.76, 0.65, 0.25, 0.15 ]  Reactances2=[2.24 0.17 0.12 1.02 0.13 0.1]  dAxisTimeConstants=Short-circuit  qAxisTimeConstants=Short-circuit  TimeConstants1="[ 4.4849  0.0681  0.1  ]"  TimeConstants2=[ 8.0, 0.03, 1.0, 0.07 ]  TimeConstants3="[  4.49  0.0681  0.0513  ]"  TimeConstants4=[ 8.0, 0.03, 0.3371, 0.0295 ]  TimeConstants5=[ 1.01, 0.053, 0.1 ]  TimeConstants6=[ 1.3201, 0.023, 1.0, 0.07 ]  TimeConstants7=[0.012 0.003 0.003]  TimeConstants8=[ 1.3201, 0.0231, 0.3371, 0.0295 ]  StatorResistance=0.037875  Mechanical=[0.1028 0.02056 2]  PolePairs=20  InitialConditions="[ 0  0  0  0  0  0  0  0  1 ]"  SetSaturation=on  Saturation=[0.6404,0.7127,0.8441,0.9214,0.9956,1.082,1.19,1.316,1.457;0.7,0.7698,0.8872,0.9466,0.9969,1.046,1.1,1.151,1.201]  LoadFlowParameters=[1,0,0,0,0]  TsPowergui=0  TsBlock=-1  IterativeModel=Trapezoidal non iterative  IterativeDiscreteModel=Trapezoidal non iterative  BusType=PV  Pref=100e6  Qref=42e6  Qmin=-inf  Qmax=inf  PLF=0  QLF=0
  Pangkalan Militer : spsThreePhaseParallelRLCLoadLib/Three-Phase Parallel RLC Load  LConnTagsString=A|B|C  Configuration=Y (grounded)  NominalVoltage=20e3  Vabc=[1e3 1e3 1e3]  Vabcp=[1e3 1e3 1e3]  NominalFrequency=50  UnbalancedPower=off  ActivePower=2.025e6  InductivePower=0.9808e6  CapacitivePower=0  Pabc=[10e3 9e3 11e3]  QLabc=[100 90 110]  QCabc=[100 90 110]  Pabcp=[10e3 9e3 11e3]  QLabcp=[100 90 110]  QCabcp=[100 90 110]  Measurements=Branch currents  LoadType=constant Z
  Pref {1..2,5..6,12..13} (6 alike) : Constant
  Pref {3..4,7..11} (7 alike) : Constant  Commented=on
  Pusat Server Data : spsThreePhaseParallelRLCLoadLib/Three-Phase Parallel RLC Load  LConnTagsString=A|B|C  Configuration=Y (grounded)  NominalVoltage=20e3  Vabc=[1e3 1e3 1e3]  Vabcp=[1e3 1e3 1e3]  NominalFrequency=50  UnbalancedPower=off  ActivePower=0.0225e6  InductivePower=0.0109e6  CapacitivePower=0  Pabc=[10e3 9e3 11e3]  QLabc=[100 90 110]  QCabc=[100 90 110]  Pabcp=[10e3 9e3 11e3]  QLabcp=[100 90 110]  QCabcp=[100 90 110]  Measurements=Branch currents  LoadType=constant Z
  Restoran dan Toko : spsThreePhaseParallelRLCLoadLib/Three-Phase Parallel RLC Load  LConnTagsString=A|B|C  Configuration=Y (grounded)  NominalVoltage=20e3  Vabc=[1e3 1e3 1e3]  Vabcp=[1e3 1e3 1e3]  NominalFrequency=50  UnbalancedPower=off  ActivePower=4.25e6  InductivePower=2.6339e6  CapacitivePower=0  Pabc=[10e3 9e3 11e3]  QLabc=[100 90 110]  QCabc=[100 90 110]  Pabcp=[10e3 9e3 11e3]  QLabcp=[100 90 110]  QCabcp=[100 90 110]  Measurements=Branch currents  LoadType=constant Z
  Rumah Sakit : spsThreePhaseParallelRLCLoadLib/Three-Phase Parallel RLC Load  LConnTagsString=A|B|C  Configuration=Y (grounded)  NominalVoltage=20e3  Vabc=[1e3 1e3 1e3]  Vabcp=[1e3 1e3 1e3]  NominalFrequency=50  UnbalancedPower=off  ActivePower=0.96e6  InductivePower=0.28e6  CapacitivePower=0  Pabc=[10e3 9e3 11e3]  QLabc=[100 90 110]  QCabc=[100 90 110]  Pabcp=[10e3 9e3 11e3]  QLabcp=[100 90 110]  QCabcp=[100 90 110]  Measurements=Branch currents  LoadType=constant Z
  Three-Phase Parallel RLC Branch{1..4} (4 alike) : spsThreePhaseParallelRLCBranchLib/Three-Phase Parallel RLC Branch  Commented=on  LConnTagsString=A|B|C  RConnTagsString=A|B|C  BranchType=RC  Resistance=1000  Inductance=1e-3  Capacitance=0.01  Measurements=None
  Three-Phase V-I Measurement : spsThreePhaseVIMeasurementLib/Three-Phase V-I Measurement  VoltageMeasurement=phase-to-ground  SetLabelV=on  LabelV=Vpltp  Vpu=off  VpuLL=off  CurrentMeasurement=yes  SetLabelI=on  LabelI=Ipltp  Ipu=off  Pbase=100e6  Vbase=500e3  OutputType=Magnitude  PhasorSimulation=off  PSBequivalent=0
  Three-Phase V-I Measurement1 : spsThreePhaseVIMeasurementLib/Three-Phase V-I Measurement  VoltageMeasurement=phase-to-ground  SetLabelV=on  LabelV=Vpltu  Vpu=off  VpuLL=off  CurrentMeasurement=yes  SetLabelI=on  LabelI=Ipltu  Ipu=off  Pbase=100e6  Vbase=500e3  OutputType=Magnitude  PhasorSimulation=off  PSBequivalent=0
  Three-Phase V-I Measurement2 : spsThreePhaseVIMeasurementLib/Three-Phase V-I Measurement  Commented=on  VoltageMeasurement=phase-to-ground  SetLabelV=on  LabelV=Vplta  Vpu=off  VpuLL=off  CurrentMeasurement=yes  SetLabelI=on  LabelI=Iplta  Ipu=off  Pbase=100e6  Vbase=500e3  OutputType=Magnitude  PhasorSimulation=off  PSBequivalent=0
  Three-Phase V-I Measurement3 : spsThreePhaseVIMeasurementLib/Three-Phase V-I Measurement  Commented=on  VoltageMeasurement=phase-to-ground  SetLabelV=on  LabelV=Vpltb  Vpu=off  VpuLL=off  CurrentMeasurement=yes  SetLabelI=on  LabelI=Ipltb  Ipu=off  Pbase=100e6  Vbase=500e3  OutputType=Magnitude  PhasorSimulation=off  PSBequivalent=0
  Three-Phase Breaker{1..13,16..17,20..32,35..36} (30 alike) : spsThreePhaseBreakerLib/Three-Phase Breaker  InitialState=closed  SwitchA=off  SwitchB=off  SwitchC=off  SwitchTimes="[0.4  1.3]"  External=off  BreakerResistance=0.01  SnubberResistance=1e6  SnubberCapacitance=inf  Measurements=None
  Three-Phase Breaker{14..15,18..19,33..34} (6 alike) : spsThreePhaseBreakerLib/Three-Phase Breaker  Commented=on  InitialState=closed  SwitchA=off  SwitchB=off  SwitchC=off  SwitchTimes="[0.4  1.3]"  External=off  BreakerResistance=0.01  SnubberResistance=1e6  SnubberCapacitance=inf  Measurements=None
  Trafo 150kV/70kV PLTA : spsThreePhaseTransformerTwoWindingsLib/Three-Phase Transformer (Two Windings)  Commented=on  Winding1Connection=Delta (D1)  Winding2Connection=Yg  CoreType=Three single-phase transformers  SetSaturation=off  Hysteresis=off  DataFile='hysteresis'  SetInitialFlux=off  Measurements=None  UNITS=pu  NominalPower=[ 1000e6 , 50 ]  Winding1=[ 150e3 , 0.005 , 0.1/(100*pi) ]  Winding2=[ 70e3 , 0.005 , 0 ]  Rm=500  Lm=500  L0=0.5  Saturation=[ 0,0 ; 0.0024,1.2 ; 1.0,1.52 ]  InitialFluxes=[ 0.8 , -0.8 , 0.7 ]  BreakLoop=off  DiscreteSolver=Trapezoidal iterative  DataType=off  TransfoNumber=1
  Trafo 150kV/70kV PLTB : spsThreePhaseTransformerTwoWindingsLib/Three-Phase Transformer (Two Windings)  Commented=on  Winding1Connection=Delta (D1)  Winding2Connection=Yg  CoreType=Three single-phase transformers  SetSaturation=off  Hysteresis=off  DataFile='hysteresis'  SetInitialFlux=off  Measurements=None  UNITS=pu  NominalPower=[ 1000e6 , 50 ]  Winding1=[ 150e3 , 0.005 , 0.1/(100*pi) ]  Winding2=[ 70e3 , 0.005 , 0 ]  Rm=500  Lm=500  L0=0.5  Saturation=[ 0,0 ; 0.0024,1.2 ; 1.0,1.52 ]  InitialFluxes=[ 0.8 , -0.8 , 0.7 ]  BreakLoop=off  DiscreteSolver=Trapezoidal iterative  DataType=off  TransfoNumber=1
  Trafo 150kV/70kV PLTP : spsThreePhaseTransformerTwoWindingsLib/Three-Phase Transformer (Two Windings)  Winding1Connection=Delta (D1)  Winding2Connection=Yg  CoreType=Three single-phase transformers  SetSaturation=off  Hysteresis=off  DataFile='hysteresis'  SetInitialFlux=off  Measurements=None  UNITS=pu  NominalPower=[ 1000e6 , 50 ]  Winding1=[ 150e3 , 0.005 , 0.1/(100*pi) ]  Winding2=[ 70e3 , 0.005 , 0 ]  Rm=500  Lm=500  L0=0.5  Saturation=[ 0,0 ; 0.0024,1.2 ; 1.0,1.52 ]  InitialFluxes=[ 0.8 , -0.8 , 0.7 ]  BreakLoop=off  DiscreteSolver=Trapezoidal iterative  DataType=off  TransfoNumber=1
  Trafo 150kV/70kV PLTU : spsThreePhaseTransformerTwoWindingsLib/Three-Phase Transformer (Two Windings)  Winding1Connection=Delta (D1)  Winding2Connection=Yg  CoreType=Three single-phase transformers  SetSaturation=off  Hysteresis=off  DataFile='hysteresis'  SetInitialFlux=off  Measurements=None  UNITS=pu  NominalPower=[ 1000e6 , 50 ]  Winding1=[ 150e3 , 0.005 , 0.1/(100*pi) ]  Winding2=[ 70e3 , 0.005 , 0 ]  Rm=500  Lm=500  L0=0.5  Saturation=[ 0,0 ; 0.0024,1.2 ; 1.0,1.52 ]  InitialFluxes=[ 0.8 , -0.8 , 0.7 ]  BreakLoop=off  DiscreteSolver=Trapezoidal iterative  DataType=off  TransfoNumber=1
  Trafo 20kV/380V Beban PubSos : spsThreePhaseTransformerTwoWindingsLib/Three-Phase Transformer (Two Windings)  Winding1Connection=Delta (D1)  Winding2Connection=Yg  CoreType=Three single-phase transformers  SetSaturation=off  Hysteresis=off  DataFile='hysteresis'  SetInitialFlux=off  Measurements=None  UNITS=pu  NominalPower=[ 1000e6 , 50 ]  Winding1=[ 20e3 , 0.005 , 0.1/(100*pi) ]  Winding2=[ 380 , 0.005 , 0 ]  Rm=500  Lm=500  L0=0.5  Saturation=[ 0,0 ; 0.0024,1.2 ; 1.0,1.52 ]  InitialFluxes=[ 0.8 , -0.8 , 0.7 ]  BreakLoop=off  DiscreteSolver=Trapezoidal iterative  DataType=off  TransfoNumber=1
  Trafo 20kV/380V Beban RT : spsThreePhaseTransformerTwoWindingsLib/Three-Phase Transformer (Two Windings)  Winding1Connection=Delta (D1)  Winding2Connection=Yg  CoreType=Three single-phase transformers  SetSaturation=off  Hysteresis=off  DataFile='hysteresis'  SetInitialFlux=off  Measurements=None  UNITS=pu  NominalPower=[ 1000e6 , 50 ]  Winding1=[ 0.95*20e3 , 0.005 , 0.1/(100*pi) ]  Winding2=[ 380 , 0.005 , 0 ]  Rm=500  Lm=500  L0=0.5  Saturation=[ 0,0 ; 0.0024,1.2 ; 1.0,1.52 ]  InitialFluxes=[ 0.8 , -0.8 , 0.7 ]  BreakLoop=off  DiscreteSolver=Trapezoidal iterative  DataType=off  TransfoNumber=1
  Trafo 20kV/70kV PLTA : spsThreePhaseTransformerTwoWindingsLib/Three-Phase Transformer (Two Windings)  Commented=on  Winding1Connection=Yg  Winding2Connection=Delta (D1)  CoreType=Three single-phase transformers  SetSaturation=off  Hysteresis=off  DataFile='hysteresis'  SetInitialFlux=off  Measurements=None  UNITS=pu  NominalPower=[ 1000e6 , 50 ]  Winding1=[ 20e3 , 0.005 , 0.1/(100*pi) ]  Winding2=[ 70e3 , 0.005 , 0 ]  Rm=500  Lm=500  L0=0.5  Saturation=[ 0,0 ; 0.0024,1.2 ; 1.0,1.52 ]  InitialFluxes=[ 0.8 , -0.8 , 0.7 ]  BreakLoop=off  DiscreteSolver=Trapezoidal iterative  DataType=off  TransfoNumber=1
  Trafo 20kV/70kV PLTB : spsThreePhaseTransformerTwoWindingsLib/Three-Phase Transformer (Two Windings)  Commented=on  Winding1Connection=Yg  Winding2Connection=Delta (D1)  CoreType=Three single-phase transformers  SetSaturation=off  Hysteresis=off  DataFile='hysteresis'  SetInitialFlux=off  Measurements=None  UNITS=pu  NominalPower=[ 1000e6 , 50 ]  Winding1=[ 20e3 , 0.005 , 0.1/(100*pi) ]  Winding2=[ 70e3 , 0.005 , 0 ]  Rm=500  Lm=500  L0=0.5  Saturation=[ 0,0 ; 0.0024,1.2 ; 1.0,1.52 ]  InitialFluxes=[ 0.8 , -0.8 , 0.7 ]  BreakLoop=off  DiscreteSolver=Trapezoidal iterative  DataType=off  TransfoNumber=1
  Trafo 20kV/70kV PLTP : spsThreePhaseTransformerTwoWindingsLib/Three-Phase Transformer (Two Windings)  Winding1Connection=Yg  Winding2Connection=Delta (D1)  CoreType=Three single-phase transformers  SetSaturation=off  Hysteresis=off  DataFile='hysteresis'  SetInitialFlux=off  Measurements=None  UNITS=pu  NominalPower=[ 1000e6 , 50 ]  Winding1=[ 20e3 , 0.005 , 0.1/(100*pi) ]  Winding2=[ 70e3 , 0.005 , 0 ]  Rm=500  Lm=500  L0=0.5  Saturation=[ 0,0 ; 0.0024,1.2 ; 1.0,1.52 ]  InitialFluxes=[ 0.8 , -0.8 , 0.7 ]  BreakLoop=off  DiscreteSolver=Trapezoidal iterative  DataType=off  TransfoNumber=1
  Trafo 20kV/70kV PLTU : spsThreePhaseTransformerTwoWindingsLib/Three-Phase Transformer (Two Windings)  Winding1Connection=Yg  Winding2Connection=Delta (D1)  CoreType=Three single-phase transformers  SetSaturation=off  Hysteresis=off  DataFile='hysteresis'  SetInitialFlux=off  Measurements=None  UNITS=pu  NominalPower=[ 1000e6 , 50 ]  Winding1=[ 20e3 , 0.005 , 0.1/(100*pi) ]  Winding2=[ 70e3 , 0.005 , 0 ]  Rm=500  Lm=500  L0=0.5  Saturation=[ 0,0 ; 0.0024,1.2 ; 1.0,1.52 ]  InitialFluxes=[ 0.8 , -0.8 , 0.7 ]  BreakLoop=off  DiscreteSolver=Trapezoidal iterative  DataType=off  TransfoNumber=1
  Trafo 70kV/150kV PLTA : spsThreePhaseTransformerTwoWindingsLib/Three-Phase Transformer (Two Windings)  Commented=on  Winding1Connection=Yg  Winding2Connection=Delta (D1)  CoreType=Three single-phase transformers  SetSaturation=off  Hysteresis=off  DataFile='hysteresis'  SetInitialFlux=off  Measurements=None  UNITS=pu  NominalPower=[ 1000e6 , 50 ]  Winding1=[ 70e3 , 0.005 , 0.1/(100*pi) ]  Winding2=[ 150e3 , 0.005 , 0 ]  Rm=500  Lm=500  L0=0.5  Saturation=[ 0,0 ; 0.0024,1.2 ; 1.0,1.52 ]  InitialFluxes=[ 0.8 , -0.8 , 0.7 ]  BreakLoop=off  DiscreteSolver=Trapezoidal iterative  DataType=off  TransfoNumber=1
  Trafo 70kV/150kV PLTB : spsThreePhaseTransformerTwoWindingsLib/Three-Phase Transformer (Two Windings)  Commented=on  Winding1Connection=Yg  Winding2Connection=Delta (D1)  CoreType=Three single-phase transformers  SetSaturation=off  Hysteresis=off  DataFile='hysteresis'  SetInitialFlux=off  Measurements=None  UNITS=pu  NominalPower=[ 1000e6 , 50 ]  Winding1=[ 70e3 , 0.005 , 0.1/(100*pi) ]  Winding2=[ 150e3 , 0.005 , 0 ]  Rm=500  Lm=500  L0=0.5  Saturation=[ 0,0 ; 0.0024,1.2 ; 1.0,1.52 ]  InitialFluxes=[ 0.8 , -0.8 , 0.7 ]  BreakLoop=off  DiscreteSolver=Trapezoidal iterative  DataType=off  TransfoNumber=1
  Trafo 70kV/150kV PLTP : spsThreePhaseTransformerTwoWindingsLib/Three-Phase Transformer (Two Windings)  Winding1Connection=Yg  Winding2Connection=Delta (D1)  CoreType=Three single-phase transformers  SetSaturation=off  Hysteresis=off  DataFile='hysteresis'  SetInitialFlux=off  Measurements=None  UNITS=pu  NominalPower=[ 1000e6 , 50 ]  Winding1=[ 70e3 , 0.005 , 0.1/(100*pi) ]  Winding2=[ 150e3 , 0.005 , 0 ]  Rm=500  Lm=500  L0=0.5  Saturation=[ 0,0 ; 0.0024,1.2 ; 1.0,1.52 ]  InitialFluxes=[ 0.8 , -0.8 , 0.7 ]  BreakLoop=off  DiscreteSolver=Trapezoidal iterative  DataType=off  TransfoNumber=1
  Trafo 70kV/150kV PLTU : spsThreePhaseTransformerTwoWindingsLib/Three-Phase Transformer (Two Windings)  Winding1Connection=Yg  Winding2Connection=Delta (D1)  CoreType=Three single-phase transformers  SetSaturation=off  Hysteresis=off  DataFile='hysteresis'  SetInitialFlux=off  Measurements=None  UNITS=pu  NominalPower=[ 1000e6 , 50 ]  Winding1=[ 70e3 , 0.005 , 0.1/(100*pi) ]  Winding2=[ 150e3 , 0.005 , 0 ]  Rm=500  Lm=500  L0=0.5  Saturation=[ 0,0 ; 0.0024,1.2 ; 1.0,1.52 ]  InitialFluxes=[ 0.8 , -0.8 , 0.7 ]  BreakLoop=off  DiscreteSolver=Trapezoidal iterative  DataType=off  TransfoNumber=1
  Trafo 70kV/20kV Gardu 1 : spsThreePhaseTransformerTwoWindingsLib/Three-Phase Transformer (Two Windings)  Winding1Connection=Delta (D1)  Winding2Connection=Yg  CoreType=Three single-phase transformers  SetSaturation=off  Hysteresis=off  DataFile='hysteresis'  SetInitialFlux=off  Measurements=None  UNITS=pu  NominalPower=[ 1000e6 , 50 ]  Winding1=[ 70e3 , 0.005 , 0.1/(100*pi) ]  Winding2=[ 20e3*1.0 , 0.005 , 0 ]  Rm=500  Lm=500  L0=0.5  Saturation=[ 0,0 ; 0.0024,1.2 ; 1.0,1.52 ]  InitialFluxes=[ 0.8 , -0.8 , 0.7 ]  BreakLoop=off  DiscreteSolver=Trapezoidal iterative  DataType=off  TransfoNumber=1
  Trafo 70kV/20kV Gardu 2 : spsThreePhaseTransformerTwoWindingsLib/Three-Phase Transformer (Two Windings)  Winding1Connection=Delta (D1)  Winding2Connection=Yg  CoreType=Three single-phase transformers  SetSaturation=off  Hysteresis=off  DataFile='hysteresis'  SetInitialFlux=off  Measurements=None  UNITS=pu  NominalPower=[ 1000e6 , 50 ]  Winding1=[ 0.975*70e3 , 0.005 , 0.1/(100*pi) ]  Winding2=[ 20e3*1.0 , 0.005 , 0 ]  Rm=500  Lm=500  L0=0.5  Saturation=[ 0,0 ; 0.0024,1.2 ; 1.0,1.52 ]  InitialFluxes=[ 0.8 , -0.8 , 0.7 ]  BreakLoop=off  DiscreteSolver=Trapezoidal iterative  DataType=off  TransfoNumber=1
  Trafo 70kV/20kV Gardu 3 : spsThreePhaseTransformerTwoWindingsLib/Three-Phase Transformer (Two Windings)  Winding1Connection=Delta (D1)  Winding2Connection=Yg  CoreType=Three single-phase transformers  SetSaturation=off  Hysteresis=off  DataFile='hysteresis'  SetInitialFlux=off  Measurements=None  UNITS=pu  NominalPower=[ 1000e6 , 50 ]  Winding1=[ 70e3 , 0.005 , 0.1/(100*pi) ]  Winding2=[ 20e3*1.0 , 0.005 , 0 ]  Rm=500  Lm=500  L0=0.5  Saturation=[ 0,0 ; 0.0024,1.2 ; 1.0,1.52 ]  InitialFluxes=[ 0.8 , -0.8 , 0.7 ]  BreakLoop=off  DiscreteSolver=Trapezoidal iterative  DataType=off  TransfoNumber=1
  Trafo 70kV/20kV Gardu 4 : spsThreePhaseTransformerTwoWindingsLib/Three-Phase Transformer (Two Windings)  Winding1Connection=Delta (D1)  Winding2Connection=Yg  CoreType=Three single-phase transformers  SetSaturation=off  Hysteresis=off  DataFile='hysteresis'  SetInitialFlux=off  Measurements=None  UNITS=pu  NominalPower=[ 1000e6 , 50 ]  Winding1=[ 70e3 , 0.005 , 0.1/(100*pi) ]  Winding2=[ 20e3*1.0 , 0.005 , 0 ]  Rm=500  Lm=500  L0=0.5  Saturation=[ 0,0 ; 0.0024,1.2 ; 1.0,1.52 ]  InitialFluxes=[ 0.8 , -0.8 , 0.7 ]  BreakLoop=off  DiscreteSolver=Trapezoidal iterative  DataType=off  TransfoNumber=1
  UKM : spsThreePhaseParallelRLCLoadLib/Three-Phase Parallel RLC Load  LConnTagsString=A|B|C  Configuration=Y (grounded)  NominalVoltage=20e3  Vabc=[1e3 1e3 1e3]  Vabcp=[1e3 1e3 1e3]  NominalFrequency=50  UnbalancedPower=off  ActivePower=5.85e6  InductivePower=2.8333e6  CapacitivePower=0  Pabc=[10e3 9e3 11e3]  QLabc=[100 90 110]  QCabc=[100 90 110]  Pabcp=[10e3 9e3 11e3]  QLabcp=[100 90 110]  QCabcp=[100 90 110]  Measurements=Branch currents  LoadType=constant Z
  Vref {1..2,5..6,12..13} (6 alike) : Constant
  Vref {3..4,7..11} (7 alike) : Constant  Commented=on
  powergui : spspowerguiLib/powergui  Priority=1  SimulationMode=Continuous  SampleTime=50e-6  frequency=60  Iterations=50  frequencyindice=60  Pbase=100e6  ErrMax=1e-4  UnitsV=kV  UnitsW=MW  buscounter=0  FunctionMessages=off  echomessages=off  EnableUseOfTLC=off  CurrentSourceSwitches=off  DisableSnubberDevices=off  DisableRonSwitches=off  DisableVfSwitches=off  DisplayEquations=off  AutomaticDiscreteSolvers=off  SolverType=Tustin/Backward Euler (TBE)  Interpol=off  ExternalGateDelay=off  methode=off  Ts=100  x0status=blocks  SPID=on  SwTol=0  HookPort=off  NonlinearTolerance=1e-4  nMaxIteration=100  ContinueOnMaxIteration=off  RestoreLinks=warning  ResistiveCurrentMeasurement=off  Frange=[0:2:500]  Ylog=off  Xlog=on  ShowGrid=off  save=off  variable=ZData  structure=0  ZoomFFT=off  StartTime=0.0  cycles=1  DisplayStyle=1  fundamental=60  FreqAxis=off  MaxFrequency=1000  frequencyindicesteady=1  RmsSteady=1  display=off
  wires:
  Bus Selector3/2 -> Excitation System 2/3  "<Stator voltage  vq (pu)>"
  Vref 1/1 -> Excitation System 1/1
  Excitation System 2/1 -> PLTU/2
  Bus Selector3/1 -> Excitation System 2/2  "<Stator voltage  vd (pu)>"
  Bus Selector1/1 -> Excitation System 1/2  "<Stator voltage  vd (pu)>"
  Excitation System 1/1 -> PLTP/2
  Pref 2/1 -> PLTU/1
  Bus Selector1/2 -> Excitation System 1/3  "<Stator voltage  vq (pu)>"
  Vref 2/1 -> Excitation System 2/1
  Pref 1/1 -> PLTP/1
  PLTU/1 -> Bus Selector3/1
  PLTP/1 -> Bus Selector1/1
  PLTA/1 -> Bus Selector2/1
  PLTB/1 -> Bus Selector4/1
  Pref 3/1 -> PLTA/1
  Vref 4/1 -> Excitation System 4/1
  Bus Selector2/2 -> Excitation System 3/3  "<Stator voltage  vq (pu)>"
  Pref 4/1 -> PLTB/1
  Excitation System 3/1 -> PLTA/2
  Bus Selector2/1 -> Excitation System 3/2  "<Stator voltage  vd (pu)>"
  Bus Selector4/1 -> Excitation System 4/2  "<Stator voltage  vd (pu)>"
  Excitation System 4/1 -> PLTB/2
  Vref 3/1 -> Excitation System 3/1
  Bus Selector4/2 -> Excitation System 4/3  "<Stator voltage  vq (pu)>"
  Vref 5/1 -> Excitation System 5/1
  Pref 5/1 -> Genset Industri/1
  Bus Selector5/1 -> Excitation System 5/2  "<Stator voltage  vd (pu)>"
  Excitation System 5/1 -> Genset Industri/2
  Bus Selector5/2 -> Excitation System 5/3  "<Stator voltage  vq (pu)>"
  Genset Industri/1 -> Bus Selector5/1
  Genset A Sekolah/1 -> Bus Selector6/1
  Bus Selector6/2 -> Excitation System 6/3  "<Stator voltage  vq (pu)>"
  Excitation System 6/1 -> Genset A Sekolah/2
  Bus Selector6/1 -> Excitation System 6/2  "<Stator voltage  vd (pu)>"
  Pref 6/1 -> Genset A Sekolah/1
  Vref 6/1 -> Excitation System 6/1
  Vref 7/1 -> Excitation System 7/1
  Pref 7/1 -> Genset B Sekolah/1
  Bus Selector7/1 -> Excitation System 7/2  "<Stator voltage  vd (pu)>"
  Excitation System 7/1 -> Genset B Sekolah/2
  Bus Selector7/2 -> Excitation System 7/3  "<Stator voltage  vq (pu)>"
  Genset B Sekolah/1 -> Bus Selector7/1
  Vref 8/1 -> Excitation System 8/1
  Pref 8/1 -> Genset C RT5/1
  Bus Selector8/1 -> Excitation System 8/2  "<Stator voltage  vd (pu)>"
  Excitation System 8/1 -> Genset C RT5/2
  Bus Selector8/2 -> Excitation System 8/3  "<Stator voltage  vq (pu)>"
  Genset C RT5/1 -> Bus Selector8/1
  Genset C RT4/1 -> Bus Selector9/1
  Bus Selector9/2 -> Excitation System 9/3  "<Stator voltage  vq (pu)>"
  Excitation System 9/1 -> Genset C RT4/2
  Bus Selector9/1 -> Excitation System 9/2  "<Stator voltage  vd (pu)>"
  Pref 9/1 -> Genset C RT4/1
  Vref 9/1 -> Excitation System 9/1
  Vref 11/1 -> Excitation System 11/1
  Pref 11/1 -> Genset B RT5/1
  Bus Selector11/1 -> Excitation System 11/2  "<Stator voltage  vd (pu)>"
  Excitation System 11/1 -> Genset B RT5/2
  Bus Selector11/2 -> Excitation System 11/3  "<Stator voltage  vq (pu)>"
  Genset B RT5/1 -> Bus Selector11/1
  Genset B RT4/1 -> Bus Selector10/1
  Bus Selector10/2 -> Excitation System 10/3  "<Stator voltage  vq (pu)>"
  Excitation System 10/1 -> Genset B RT4/2
  Bus Selector10/1 -> Excitation System 10/2  "<Stator voltage  vd (pu)>"
  Pref 10/1 -> Genset B RT4/1
  Vref 10/1 -> Excitation System 10/1
  Vref 13/1 -> Excitation System 13/1
  Pref 13/1 -> Genset A RT5/1
  Bus Selector13/1 -> Excitation System 13/2  "<Stator voltage  vd (pu)>"
  Excitation System 13/1 -> Genset A RT5/2
  Bus Selector13/2 -> Excitation System 13/3  "<Stator voltage  vq (pu)>"
  Genset A RT5/1 -> Bus Selector13/1
  Genset A RT4/1 -> Bus Selector12/1
  Bus Selector12/2 -> Excitation System 12/3  "<Stator voltage  vq (pu)>"
  Excitation System 12/1 -> Genset A RT4/2
  Bus Selector12/1 -> Excitation System 12/2  "<Stator voltage  vd (pu)>"
  Pref 12/1 -> Genset A RT4/1
  Vref 12/1 -> Excitation System 12/1
  connections:
  Three-Phase Parallel RLC Branch2/RConn3 -- Three-Phase Parallel RLC Branch2/RConn2 -- Three-Phase Parallel RLC Branch2/RConn1 -- Ground1/LConn1
  Three-Phase Parallel RLC Branch1/RConn1 -- Three-Phase Parallel RLC Branch1/RConn2 -- Three-Phase Parallel RLC Branch1/RConn3 -- Ground/LConn1
  Three-Phase V-I Measurement1/LConn2 -- PLTU/RConn2 -- Three-Phase Parallel RLC Branch2/LConn2
  Three-Phase V-I Measurement/LConn3 -- PLTP/RConn3 -- Three-Phase Parallel RLC Branch1/LConn3
  Three-Phase V-I Measurement/LConn2 -- PLTP/RConn2 -- Three-Phase Parallel RLC Branch1/LConn2
  Three-Phase V-I Measurement/LConn1 -- PLTP/RConn1 -- Three-Phase Parallel RLC Branch1/LConn1
  Three-Phase V-I Measurement1/LConn3 -- PLTU/RConn3 -- Three-Phase Parallel RLC Branch2/LConn3
  Three-Phase V-I Measurement1/LConn1 -- PLTU/RConn1 -- Three-Phase Parallel RLC Branch2/LConn1
  Ground3/LConn1 -- Three-Phase Parallel RLC Branch4/RConn3 -- Three-Phase Parallel RLC Branch4/RConn1 -- Three-Phase Parallel RLC Branch4/RConn2
  Ground2/LConn1 -- Three-Phase Parallel RLC Branch3/RConn1 -- Three-Phase Parallel RLC Branch3/RConn3 -- Three-Phase Parallel RLC Branch3/RConn2
  Three-Phase Parallel RLC Branch4/LConn2 -- PLTB/RConn2 -- Three-Phase V-I Measurement3/LConn2
  PLTA/RConn3 -- Three-Phase Parallel RLC Branch3/LConn3 -- Three-Phase V-I Measurement2/LConn3
  PLTA/RConn2 -- Three-Phase Parallel RLC Branch3/LConn2 -- Three-Phase V-I Measurement2/LConn2
  PLTA/RConn1 -- Three-Phase Parallel RLC Branch3/LConn1 -- Three-Phase V-I Measurement2/LConn1
  Three-Phase Parallel RLC Branch4/LConn3 -- PLTB/RConn3 -- Three-Phase V-I Measurement3/LConn3
  Three-Phase Parallel RLC Branch4/LConn1 -- PLTB/RConn1 -- Three-Phase V-I Measurement3/LConn1
  Trafo 70kV/150kV PLTB/RConn1 -- Three-Phase Breaker15/LConn1
  Trafo 70kV/150kV PLTB/RConn2 -- Three-Phase Breaker15/LConn2
  Trafo 70kV/150kV PLTB/RConn3 -- Three-Phase Breaker15/LConn3
  Line PLTB/LConn1 -- Three-Phase Breaker15/RConn1
  Line PLTB/LConn2 -- Three-Phase Breaker15/RConn2
  Line PLTB/LConn3 -- Three-Phase Breaker15/RConn3
  Trafo 70kV/150kV PLTA/RConn1 -- Three-Phase Breaker14/LConn1
  Trafo 70kV/150kV PLTA/RConn2 -- Three-Phase Breaker14/LConn2
  Trafo 70kV/150kV PLTA/RConn3 -- Three-Phase Breaker14/LConn3
  Line PLTA/LConn1 -- Three-Phase Breaker14/RConn1
  Line PLTA/LConn2 -- Three-Phase Breaker14/RConn2
  Line PLTA/LConn3 -- Three-Phase Breaker14/RConn3
  Trafo 70kV/150kV PLTU/RConn1 -- Three-Phase Breaker13/LConn1
  Trafo 70kV/150kV PLTU/RConn2 -- Three-Phase Breaker13/LConn2
  Trafo 70kV/150kV PLTU/RConn3 -- Three-Phase Breaker13/LConn3
  Line PLTU/LConn1 -- Three-Phase Breaker13/RConn1
  Line PLTU/LConn2 -- Three-Phase Breaker13/RConn2
  Line PLTU/LConn3 -- Three-Phase Breaker13/RConn3
  Trafo 70kV/150kV PLTP/RConn1 -- Three-Phase Breaker35/LConn1 -- Three-Phase Breaker12/LConn1
  Trafo 70kV/150kV PLTP/RConn2 -- Three-Phase Breaker35/LConn2 -- Three-Phase Breaker12/LConn2
  Trafo 70kV/150kV PLTP/RConn3 -- Three-Phase Breaker35/LConn3 -- Three-Phase Breaker12/LConn3
  Line PLTP/LConn1 -- Three-Phase Breaker12/RConn1
  Line PLTP/LConn2 -- Three-Phase Breaker12/RConn2
  Line PLTP/LConn3 -- Three-Phase Breaker12/RConn3
  Line PLTP/RConn1 -- Three-Phase Breaker16/LConn1
  Line PLTP/RConn2 -- Three-Phase Breaker16/LConn2
  Line PLTP/RConn3 -- Three-Phase Breaker16/LConn3
  Line PLTU/RConn1 -- Three-Phase Breaker17/LConn1
  Line PLTU/RConn2 -- Three-Phase Breaker17/LConn2
  Line PLTU/RConn3 -- Three-Phase Breaker17/LConn3
  Line PLTA/RConn1 -- Three-Phase Breaker18/LConn1
  Line PLTA/RConn2 -- Three-Phase Breaker18/LConn2
  Line PLTA/RConn3 -- Three-Phase Breaker18/LConn3
  Line PLTB/RConn1 -- Three-Phase Breaker19/LConn1
  Line PLTB/RConn2 -- Three-Phase Breaker19/LConn2
  Line PLTB/RConn3 -- Three-Phase Breaker19/LConn3
  Line Gardu 1-2/LConn3 -- Three-Phase Breaker4/RConn3
  Line Gardu 1-2/RConn2 -- Three-Phase Breaker5/LConn2
  Line Gardu 1-2/RConn1 -- Three-Phase Breaker5/LConn1
  Line Gardu 1-2/RConn3 -- Three-Phase Breaker5/LConn3
  Line Gardu 1-2/LConn1 -- Three-Phase Breaker4/RConn1
  Line Gardu 1-2/LConn2 -- Three-Phase Breaker4/RConn2
  Three-Phase Breaker16/RConn1 -- Three-Phase Breaker36/RConn1 -- Trafo 150kV/70kV PLTP/LConn1
  Three-Phase Breaker16/RConn2 -- Three-Phase Breaker36/RConn2 -- Trafo 150kV/70kV PLTP/LConn2
  Three-Phase Breaker16/RConn3 -- Three-Phase Breaker36/RConn3 -- Trafo 150kV/70kV PLTP/LConn3
  Trafo 150kV/70kV PLTU/LConn1 -- Three-Phase Breaker17/RConn1
  Trafo 150kV/70kV PLTU/LConn2 -- Three-Phase Breaker17/RConn2
  Trafo 150kV/70kV PLTU/LConn3 -- Three-Phase Breaker17/RConn3
  Trafo 150kV/70kV PLTA/LConn1 -- Three-Phase Breaker18/RConn1
  Trafo 150kV/70kV PLTA/LConn2 -- Three-Phase Breaker18/RConn2
  Trafo 150kV/70kV PLTA/LConn3 -- Three-Phase Breaker18/RConn3
  Trafo 150kV/70kV PLTB/LConn1 -- Three-Phase Breaker19/RConn1
  Trafo 150kV/70kV PLTB/LConn2 -- Three-Phase Breaker19/RConn2
  Trafo 150kV/70kV PLTB/LConn3 -- Three-Phase Breaker19/RConn3
  Line Gardu 2-3/LConn2 -- Three-Phase Breaker6/RConn2
  Line Gardu 2-3/LConn1 -- Three-Phase Breaker6/RConn1
  Line Gardu 2-3/RConn1 -- Three-Phase Breaker7/LConn1
  Line Gardu 2-3/RConn2 -- Three-Phase Breaker7/LConn2
  Line Gardu 2-3/RConn3 -- Three-Phase Breaker7/LConn3
  Line Gardu 2-3/LConn3 -- Three-Phase Breaker6/RConn3
  Line Gardu 3-4/LConn3 -- Three-Phase Breaker8/RConn3
  Line Gardu 3-4/RConn3 -- Three-Phase Breaker9/LConn3
  Line Gardu 3-4/RConn1 -- Three-Phase Breaker9/LConn1
  Line Gardu 3-4/RConn2 -- Three-Phase Breaker9/LConn2
  Line Gardu 3-4/LConn1 -- Three-Phase Breaker8/RConn1
  Line Gardu 3-4/LConn2 -- Three-Phase Breaker8/RConn2
  Three-Phase Breaker7/RConn2 -- Three-Phase Breaker4/LConn2 -- Three-Phase Breaker2/LConn2 -- Trafo 150kV/70kV PLTU/RConn2 -- Three-Phase Breaker24/RConn2
  Three-Phase Breaker7/RConn3 -- Three-Phase Breaker4/LConn3 -- Three-Phase Breaker2/LConn3 -- Trafo 150kV/70kV PLTU/RConn3 -- Three-Phase Breaker24/RConn3
  Line Gardu 1-3/LConn2 -- Three-Phase Breaker10/RConn2
  Line Gardu 1-3/LConn1 -- Three-Phase Breaker10/RConn1
  Line Gardu 1-3/RConn1 -- Three-Phase Breaker11/LConn1
  Line Gardu 1-3/RConn2 -- Three-Phase Breaker11/LConn2
  Line Gardu 1-3/RConn3 -- Three-Phase Breaker11/LConn3
  Line Gardu 1-3/LConn3 -- Three-Phase Breaker10/RConn3
  Line Gardu 1-4/LConn3 -- Three-Phase Breaker21/RConn3
  Line Gardu 1-4/RConn3 -- Three-Phase Breaker22/LConn3
  Line Gardu 1-4/RConn1 -- Three-Phase Breaker22/LConn1
  Line Gardu 1-4/LConn1 -- Three-Phase Breaker21/RConn1
  Line Gardu 1-4/RConn2 -- Three-Phase Breaker22/LConn2
  Line Gardu 1-4/LConn2 -- Three-Phase Breaker21/RConn2
  Line Gardu 2-4/LConn1 -- Three-Phase Breaker23/RConn1
  Line Gardu 2-4/RConn1 -- Three-Phase Breaker24/LConn1
  Line Gardu 2-4/RConn2 -- Three-Phase Breaker24/LConn2
  Line Gardu 2-4/RConn3 -- Three-Phase Breaker24/LConn3
  Line Gardu 2-4/LConn3 -- Three-Phase Breaker23/RConn3
  Line Gardu 2-4/LConn2 -- Three-Phase Breaker23/RConn2
  Three-Phase Breaker7/RConn1 -- Three-Phase Breaker4/LConn1 -- Three-Phase Breaker2/LConn1 -- Trafo 150kV/70kV PLTU/RConn1 -- Three-Phase Breaker24/RConn1
  Trafo 150kV/70kV PLTP/RConn1 -- Three-Phase Breaker22/RConn1 -- Three-Phase Breaker11/RConn1 -- Three-Phase Breaker1/LConn1 -- Three-Phase Breaker5/RConn1
  Trafo 150kV/70kV PLTP/RConn2 -- Three-Phase Breaker22/RConn2 -- Three-Phase Breaker11/RConn2 -- Three-Phase Breaker1/LConn2 -- Three-Phase Breaker5/RConn2
  Trafo 150kV/70kV PLTP/RConn3 -- Three-Phase Breaker22/RConn3 -- Three-Phase Breaker11/RConn3 -- Three-Phase Breaker1/LConn3 -- Three-Phase Breaker5/RConn3
  Three-Phase Breaker10/LConn1 -- Trafo 150kV/70kV PLTA/RConn1 -- Three-Phase Breaker6/LConn1 -- Three-Phase Breaker9/RConn1 -- Three-Phase Breaker3/LConn1
  Three-Phase Breaker10/LConn2 -- Trafo 150kV/70kV PLTA/RConn2 -- Three-Phase Breaker9/RConn2 -- Three-Phase Breaker3/LConn2 -- Three-Phase Breaker6/LConn2
  Three-Phase Breaker10/LConn3 -- Trafo 150kV/70kV PLTA/RConn3 -- Three-Phase Breaker9/RConn3 -- Three-Phase Breaker3/LConn3 -- Three-Phase Breaker6/LConn3
  Three-Phase Breaker21/LConn1 -- Trafo 150kV/70kV PLTB/RConn1 -- Three-Phase Breaker26/LConn1 -- Three-Phase Breaker8/LConn1 -- Three-Phase Breaker23/LConn1
  Three-Phase Breaker21/LConn2 -- Trafo 150kV/70kV PLTB/RConn2 -- Three-Phase Breaker26/LConn2 -- Three-Phase Breaker8/LConn2 -- Three-Phase Breaker23/LConn2
  Three-Phase Breaker8/LConn3 -- Three-Phase Breaker26/LConn3 -- Three-Phase Breaker23/LConn3 -- Trafo 150kV/70kV PLTB/RConn3 -- Three-Phase Breaker21/LConn3
  Beban B RT4/LConn1 -- Genset B RT4/RConn1
  Trafo 20kV/380V Beban RT/RConn2 -- Beban B RT2/LConn2 -- Beban B RT1/LConn2 -- Beban B RT3/LConn2 -- Beban A RT3/LConn2 -- Beban A RT2/LConn2 -- Beban A RT1/LConn2 -- Beban C RT1/LConn2 -- Beban C RT2/LConn2 -- Beban C RT3/LConn2
  Beban B RT2/LConn3 -- Beban B RT1/LConn3 -- Beban B RT3/LConn3 -- Beban A RT3/LConn3 -- Beban A RT2/LConn3 -- Beban A RT1/LConn3 -- Beban C RT1/LConn3 -- Beban C RT2/LConn3 -- Beban C RT3/LConn3 -- Trafo 20kV/380V Beban RT/RConn3
  Line Beban RT/RConn2 -- Three-Phase Breaker25/LConn2
  Line Beban RT/RConn1 -- Three-Phase Breaker25/LConn1
  Line Beban RT/LConn3 -- Three-Phase Breaker20/RConn3
  Line Beban RT/LConn1 -- Three-Phase Breaker20/RConn1
  Line Beban RT/LConn2 -- Three-Phase Breaker20/RConn2
  Line Beban RT/RConn3 -- Three-Phase Breaker25/LConn3
  Three-Phase Breaker25/RConn1 -- Three-Phase Breaker30/RConn1 -- Trafo 20kV/380V Beban RT/LConn1
  Three-Phase Breaker25/RConn2 -- Three-Phase Breaker30/RConn2 -- Trafo 20kV/380V Beban RT/LConn2
  Three-Phase Breaker25/RConn3 -- Trafo 20kV/380V Beban RT/LConn3 -- Three-Phase Breaker30/RConn3
  Three-Phase Breaker1/RConn1 -- Trafo 70kV/20kV Gardu 1/LConn1
  Three-Phase Breaker1/RConn2 -- Trafo 70kV/20kV Gardu 1/LConn2
  Three-Phase Breaker1/RConn3 -- Trafo 70kV/20kV Gardu 1/LConn3
  Trafo 70kV/20kV Gardu 2/LConn2 -- Three-Phase Breaker2/RConn2
  Trafo 70kV/20kV Gardu 2/LConn1 -- Three-Phase Breaker2/RConn1
  Trafo 70kV/20kV Gardu 2/LConn3 -- Three-Phase Breaker2/RConn3
  Trafo 70kV/20kV Gardu 4/LConn3 -- Three-Phase Breaker26/RConn3
  Trafo 70kV/20kV Gardu 4/LConn1 -- Three-Phase Breaker26/RConn1
  Trafo 70kV/20kV Gardu 4/LConn2 -- Three-Phase Breaker26/RConn2
  Trafo 70kV/20kV Gardu 3/LConn3 -- Three-Phase Breaker3/RConn3
  Trafo 70kV/20kV Gardu 3/LConn1 -- Three-Phase Breaker3/RConn1
  Trafo 70kV/20kV Gardu 3/LConn2 -- Three-Phase Breaker3/RConn2
  Mall dan Hotel/LConn1 -- Restoran dan Toko/LConn1 -- Genset Industri/RConn1 -- Industri Kecil/LConn1 -- Industri Sedang/LConn1 -- Industri Besar/LConn1 -- UKM/LConn1
  Mall dan Hotel/LConn2 -- Restoran dan Toko/LConn2 -- Genset Industri/RConn2 -- Industri Kecil/LConn2 -- Industri Sedang/LConn2 -- Industri Besar/LConn2 -- UKM/LConn2
  Mall dan Hotel/LConn3 -- Restoran dan Toko/LConn3 -- Genset Industri/RConn3 -- UKM/LConn3 -- Industri Kecil/LConn3 -- Industri Sedang/LConn3 -- Industri Besar/LConn3
  Istana Negara/LConn1 -- Trafo 70kV/20kV Gardu 3/RConn1 -- Rumah Sakit/LConn1 -- Pusat Server Data/LConn1 -- Kantor Lembaga Data/LConn1 -- Pangkalan Militer/LConn1
  Istana Negara/LConn2 -- Trafo 70kV/20kV Gardu 3/RConn2 -- Rumah Sakit/LConn2 -- Pusat Server Data/LConn2 -- Kantor Lembaga Data/LConn2 -- Pangkalan Militer/LConn2
  Istana Negara/LConn3 -- Trafo 70kV/20kV Gardu 3/RConn3 -- Rumah Sakit/LConn3 -- Pusat Server Data/LConn3 -- Kantor Lembaga Data/LConn3 -- Pangkalan Militer/LConn3
  Trafo 70kV/20kV Gardu 4/RConn2 -- Three-Phase Breaker27/LConn2
  Trafo 70kV/20kV Gardu 4/RConn3 -- Three-Phase Breaker27/LConn3
  Trafo 20kV/380V Beban PubSos/LConn1 -- Three-Phase Breaker28/RConn1
  Line Beban PubSos/LConn3 -- Three-Phase Breaker27/RConn3
  Line Beban PubSos/LConn2 -- Three-Phase Breaker27/RConn2
  Line Beban PubSos/LConn1 -- Three-Phase Breaker27/RConn1
  Trafo 20kV/380V Beban PubSos/LConn2 -- Three-Phase Breaker28/RConn2
  Line Beban PubSos/RConn1 -- Three-Phase Breaker28/LConn1
  Trafo 20kV/380V Beban PubSos/LConn3 -- Three-Phase Breaker28/RConn3
  Line Beban PubSos/RConn2 -- Three-Phase Breaker28/LConn2
  Line Beban PubSos/RConn3 -- Three-Phase Breaker28/LConn3
  Trafo 70kV/20kV Gardu 4/RConn1 -- Three-Phase Breaker27/LConn1
  Beban B Penerangan Jalan Umum/LConn1 -- Beban B Rumah Ibadah/LConn1 -- Trafo 20kV/380V Beban PubSos/RConn1 -- Beban C Rumah Ibadah/LConn1 -- Beban C Penerangan Jalan Umum/LConn1 -- Beban C Sekolah dan Universitas/LConn1 -- Beban A Penerangan Jalan Umum/LConn1 -- Beban A Rumah Ibadah/LConn1
  Genset B Sekolah/RConn2 -- Beban B Sekolah dan Universitas/LConn2
  Beban A Sekolah dan Universitas/LConn3 -- Genset A Sekolah/RConn3
  Three-Phase V-I Measurement/RConn1 -- Trafo 20kV/70kV PLTP/LConn1
  Three-Phase V-I Measurement/RConn2 -- Trafo 20kV/70kV PLTP/LConn2
  Three-Phase V-I Measurement/RConn3 -- Trafo 20kV/70kV PLTP/LConn3
  Three-Phase V-I Measurement2/RConn1 -- Trafo 20kV/70kV PLTA/LConn1
  Three-Phase V-I Measurement2/RConn2 -- Trafo 20kV/70kV PLTA/LConn2
  Three-Phase V-I Measurement2/RConn3 -- Trafo 20kV/70kV PLTA/LConn3
  Three-Phase V-I Measurement3/RConn1 -- Trafo 20kV/70kV PLTB/LConn1
  Three-Phase V-I Measurement3/RConn2 -- Trafo 20kV/70kV PLTB/LConn2
  Three-Phase V-I Measurement3/RConn3 -- Trafo 20kV/70kV PLTB/LConn3
  Three-Phase V-I Measurement1/RConn1 -- Trafo 20kV/70kV PLTU/LConn1
  Three-Phase V-I Measurement1/RConn2 -- Trafo 20kV/70kV PLTU/LConn2
  Three-Phase V-I Measurement1/RConn3 -- Trafo 20kV/70kV PLTU/LConn3
  Trafo 70kV/20kV Gardu 1/RConn1 -- Three-Phase Breaker29/LConn1 -- Three-Phase Breaker20/LConn1
  Trafo 70kV/20kV Gardu 1/RConn2 -- Three-Phase Breaker29/LConn2 -- Three-Phase Breaker20/LConn2
  Trafo 70kV/20kV Gardu 1/RConn3 -- Three-Phase Breaker29/LConn3 -- Three-Phase Breaker20/LConn3
  Line Beban RT1/LConn1 -- Three-Phase Breaker29/RConn1
  Line Beban RT1/LConn3 -- Three-Phase Breaker29/RConn3
  Line Beban RT1/LConn2 -- Three-Phase Breaker29/RConn2
  Line Beban RT1/RConn1 -- Three-Phase Breaker30/LConn1
  Line Beban RT1/RConn3 -- Three-Phase Breaker30/LConn3
  Line Beban RT1/RConn2 -- Three-Phase Breaker30/LConn2
  Trafo 20kV/70kV PLTP/RConn1 -- Three-Phase Breaker31/LConn1
  Trafo 20kV/70kV PLTP/RConn2 -- Three-Phase Breaker31/LConn2
  Trafo 20kV/70kV PLTP/RConn3 -- Three-Phase Breaker31/LConn3
  Three-Phase Breaker31/RConn1 -- Trafo 70kV/150kV PLTP/LConn1
  Three-Phase Breaker31/RConn2 -- Trafo 70kV/150kV PLTP/LConn2
  Three-Phase Breaker31/RConn3 -- Trafo 70kV/150kV PLTP/LConn3
  Trafo 20kV/70kV PLTU/RConn1 -- Three-Phase Breaker32/LConn1
  Trafo 20kV/70kV PLTU/RConn2 -- Three-Phase Breaker32/LConn2
  Trafo 20kV/70kV PLTU/RConn3 -- Three-Phase Breaker32/LConn3
  Three-Phase Breaker32/RConn1 -- Trafo 70kV/150kV PLTU/LConn1
  Three-Phase Breaker32/RConn2 -- Trafo 70kV/150kV PLTU/LConn2
  Three-Phase Breaker32/RConn3 -- Trafo 70kV/150kV PLTU/LConn3
  Trafo 20kV/70kV PLTA/RConn1 -- Three-Phase Breaker33/LConn1
  Trafo 20kV/70kV PLTA/RConn2 -- Three-Phase Breaker33/LConn2
  Trafo 20kV/70kV PLTA/RConn3 -- Three-Phase Breaker33/LConn3
  Three-Phase Breaker33/RConn1 -- Trafo 70kV/150kV PLTA/LConn1
  Three-Phase Breaker33/RConn2 -- Trafo 70kV/150kV PLTA/LConn2
  Three-Phase Breaker33/RConn3 -- Trafo 70kV/150kV PLTA/LConn3
  Trafo 20kV/70kV PLTB/RConn1 -- Three-Phase Breaker34/LConn1
  Trafo 20kV/70kV PLTB/RConn2 -- Three-Phase Breaker34/LConn2
  Trafo 20kV/70kV PLTB/RConn3 -- Three-Phase Breaker34/LConn3
  Three-Phase Breaker34/RConn1 -- Trafo 70kV/150kV PLTB/LConn1
  Three-Phase Breaker34/RConn2 -- Trafo 70kV/150kV PLTB/LConn2
  Three-Phase Breaker34/RConn3 -- Trafo 70kV/150kV PLTB/LConn3
  Line PLTP1/RConn3 -- Three-Phase Breaker36/LConn3
  Line PLTP1/LConn3 -- Three-Phase Breaker35/RConn3
  Three-Phase Breaker35/RConn1 -- Line PLTP1/LConn1
  Line PLTP1/RConn1 -- Three-Phase Breaker36/LConn1
  Three-Phase Breaker36/LConn2 -- Line PLTP1/RConn2
  Line PLTP1/LConn2 -- Three-Phase Breaker35/RConn2
  Beban C RT4/LConn2 -- Genset C RT4/RConn2
  Beban C RT4/LConn3 -- Genset C RT4/RConn3
  Beban C RT4/LConn1 -- Genset C RT4/RConn1
  Beban C RT5/LConn2 -- Genset C RT5/RConn2
  Beban C RT5/LConn3 -- Genset C RT5/RConn3
  Beban C RT5/LConn1 -- Genset C RT5/RConn1
  Beban B RT5/LConn2 -- Genset B RT5/RConn2
  Beban B RT4/LConn2 -- Genset B RT4/RConn2
  Beban B RT5/LConn3 -- Genset B RT5/RConn3
  Beban B RT4/LConn3 -- Genset B RT4/RConn3
  Trafo 20kV/380V Beban RT/RConn1 -- Beban B RT2/LConn1 -- Beban B RT1/LConn1 -- Beban B RT3/LConn1 -- Beban A RT3/LConn1 -- Beban A RT2/LConn1 -- Beban A RT1/LConn1 -- Beban C RT1/LConn1 -- Beban C RT2/LConn1 -- Beban C RT3/LConn1
  Beban B RT5/LConn1 -- Genset B RT5/RConn1
  Beban A RT4/LConn1 -- Genset A RT4/RConn1
  Beban A RT5/LConn1 -- Genset A RT5/RConn1
  Beban A RT4/LConn2 -- Genset A RT4/RConn2
  Beban A RT5/LConn2 -- Genset A RT5/RConn2
  Beban A RT4/LConn3 -- Genset A RT4/RConn3
  Beban A RT5/LConn3 -- Genset A RT5/RConn3
  Genset B Sekolah/RConn1 -- Beban B Sekolah dan Universitas/LConn1
  Genset B Sekolah/RConn3 -- Beban B Sekolah dan Universitas/LConn3
  Trafo 20kV/380V Beban PubSos/RConn2 -- Beban B Penerangan Jalan Umum/LConn2 -- Beban B Rumah Ibadah/LConn2 -- Beban C Rumah Ibadah/LConn2 -- Beban C Penerangan Jalan Umum/LConn2 -- Beban C Sekolah dan Universitas/LConn2 -- Beban A Penerangan Jalan Umum/LConn2 -- Beban A Rumah Ibadah/LConn2
  Beban A Sekolah dan Universitas/LConn1 -- Genset A Sekolah/RConn1
  Beban A Sekolah dan Universitas/LConn2 -- Genset A Sekolah/RConn2
  Beban B Penerangan Jalan Umum/LConn3 -- Beban B Rumah Ibadah/LConn3 -- Trafo 20kV/380V Beban PubSos/RConn3 -- Beban C Rumah Ibadah/LConn3 -- Beban C Penerangan Jalan Umum/LConn3 -- Beban C Sekolah dan Universitas/LConn3 -- Beban A Penerangan Jalan Umum/LConn3 -- Beban A Rumah Ibadah/LConn3
